simulink model "x64_15l_gonly"  (R2012b)
settings: Solver=VariableStepDiscrete  SolverMode=SingleTasking  StartTime=0.0  StopTime=10.0  RelTol=1e-3
undefined symbols (not defined in the file): gcbh, pfb_coeff_gen_calc, ROACH, xlBlockLoadCallback
libraries: xbsIndex_r4 x10760, casper_library_misc x122, casper_library_delays x52, ox_lib x14, xrbsComm_r4 x8, xps_library x8
(part 1 of 128)
settings Model: Creator=root  LastModifiedBy=jack
settings DataIOCC: SignalLoggingSaveFormat=ModelDataLogs
settings OptimizationCC: InlineParams=on
settings DebuggingCC: FcnCallInpInsideContextMsg=UseLocalSettings  StrictBusMsg=Warning
settings GRTTargetCC: CombineOutputUpdateFcns=off  GRTInterface=on

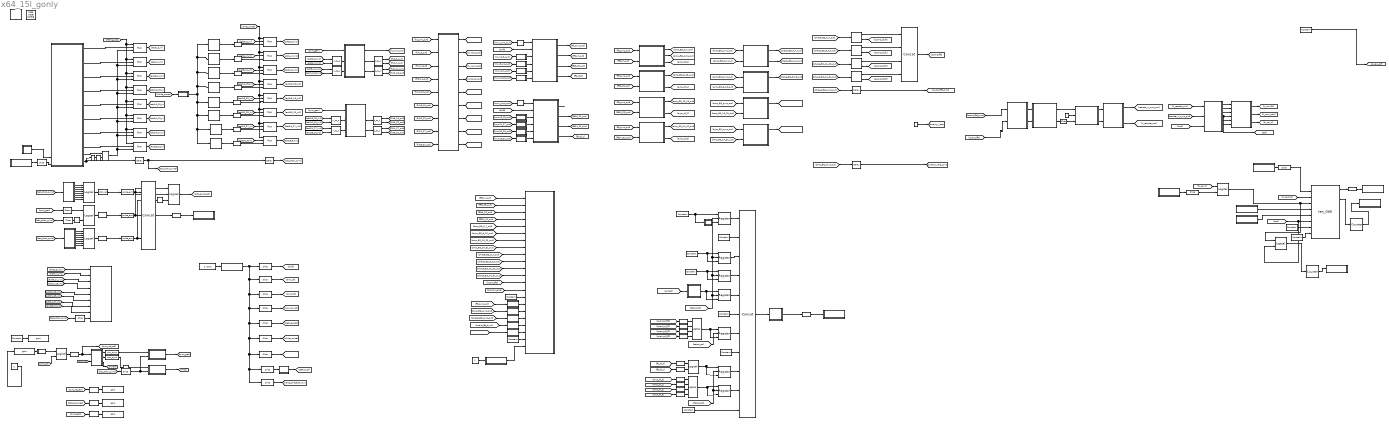
== system x64_15l_gonly ==
  note: revision history:
      |
      | r021a: updated ADC, PFB, FFT blocks
      | removed BF XAUI and logic
      | r021b: get rid of stupid FFTT subsystem
  note: The adc_sync_test reg allows the
      | user to confirm that all 8 ADC chips
      | are syncing together, and that these
      | ADC syncs are arriving the clock before
      | the master sync.
      | If all is going well, the register should
      | show one
  note: bits 0-10: shift
  note: bit 13: xaui tx enable trig
  note: bit 11: sync arm
  note: bit 12: sync rst
  note: We tag on some logic after the
      | sync gen to ensure that a sync pulse
      | arrives the clock before the adc_channel
      | sync, which signifies the arrival
      | of the first multiplexed channel on the
      | adc lines
  note: bit 14: mux in adc chans 4-7 for debug
  note: Data is reordered so that an entire window
      | can be shifted through the FFT
  note: After the FFT, each signal now carries spectra from 8
      | consecutive ADC channels
  note: NFFT = 11
      |
      | NFFT/2 channels
      | 32 (=2^5) ants
      |
      | => 2^(NFFT+4) coeffs
      |
      | 4=2^2 simultaneous streams
      | => 2^(NFFT+2) coeffs per stream
  note: We equalise amplitude and
      | pass data to be quantized to
      | 4 bits and sent to the X engine
      | over XAUI
      | 18 bit precision is maintained so that
      | phase corrections can be added to the
      | data stream going to the fft imaging system.
  note: Phase corrections to the non-FX correlator
      | data streams are implemented here, before quantization
      | to 4 bits takes place
  note: This is the order that will be used by the beamformer+fftt
      | A single freq. channel is repeated  2^(QDR_output_blocksize - 3) times
  note: Whilst the X engine expects groups of a single channel and a single
      | antenna, the fourier imager expects blocks of all antennas * one frequency channel.
  note: [ [0:8:1023] [1:8:1023] [2:8:1023] [3:8:1023]
      | [4:8:1023] [5:8:1023] [6:8:1023] [7:8:1023] ]
  note: Data is tagged with a mcnt number and sync and eof headers.
      | These are later decoded and used for error checking / data ordering
      | in the spatial imager and X-engines
  note: r022a: added MCNT sw reg, compile for library with xBlock SW reg
      | r022b: added white noise generators
      |
      | r023a: 14/03/2011 Changed ADC sync test flags to pulse extend rather than periodically
      | reset registers. Replaced of_reg and snap blocks with status reg from GMRT F-engine
      | and multipurpose snap block from GMRT F-engine. Changed adc power block for power/snap combination.
      | Changed sync period to take into account non 2^N reorder orders in various blocks.
      | 15/03/2011 Black boxed FIR/FFT. Various syntax fixes
  note: bit 15: white noise generator
  note: bit 15: white noise generator rst
  note: ADC overflow
      | Beam Buffer write clash
      | Beam Buffer bad
      | beam buffer valid
      | sync armed
      | beam coeff of
      | fft overflow
      | amp eq overflow
  note: Non 2^N periods:
      | fft mux -- 13
      | QDR transpose -- 11
      | post QDR reorder -- 10
      | reorder 1_ant_a_time -- 7
      | LCM(13,11,10,7) = 10010
  note: bit 19: reset status flags
  note: The FFT interleaves antenna spectra (though blocks of N_FFT/2 channels
      | remain contiguous.
      | The signal description "0_7" here, means the first 7 antennas, in the order:
      | 0,4,1,5,2,6,3,7
      | Similarly, signals named "x_x+7" have the order
      | x,x+4,x+1,x+5,x+2,x+6,x+3,x+7
      | This order needs to be reflected in the arrangement of coefficients
      | in the downstream EQ RAM blocks.
  note: bit 20: Xengine phased input mux
  note: scale inputs down by 2 bits
  " System Generator" : xbsIndex_r4/ System Generator  Tag=genX  xilinxfamily=virtex5  part=xc5vsx95t  speed=-1  package=ff1136  synthesis_tool=XST  clock_wrapper=Clock Enables  directory=./x64_32f_024i_15lg/sysgen  proj_type=Project Navigator  Synth_file=XST Defaults  Impl_file=ISE Defaults  testbench=off  simulink_period=1  sysclk_period=6.25  dcm_input_clock_period=100  incr_netlist=off  trim_vbits=Everywhere in SubSystem  dbl_ovrd=According to Block Masks  core_generation=According to Block Masks  run_coregen=off  deprecated_control=off  eval_field=0  block_type=sysgen
      settings: block_version=11.4
  Concat1 : xbsIndex_r4/Concat  num_inputs=11  dbl_ovrd=off  block_type=concat
  Concat4 : xbsIndex_r4/Concat  num_inputs=4  dbl_ovrd=off  block_type=concat
  Concat6 : xbsIndex_r4/Concat  num_inputs=3  dbl_ovrd=off  block_type=concat
  Constant : xbsIndex_r4/Constant  const=1  gui_display_data_type=Fixed-point  arith_type=Boolean  n_bits=16  bin_pt=14  preci_type=Single  exp_width=8  frac_width=24  explicit_period=on  period=1  equ=P=C  opselect=C  inp2=PCIN>>17  opr=+  inp1=P  carry=CIN  dbl_ovrd=off  block_type=constant
      settings: block_version=11.4
  Constant1 : xbsIndex_r4/Constant  const=0  gui_display_data_type=Fixed-point  arith_type=Signed (2's comp)  n_bits=32  bin_pt=0  preci_type=Single  exp_width=8  frac_width=24  explicit_period=on  period=1  equ=P=C  opselect=C  inp2=PCIN>>17  opr=+  inp1=P  carry=CIN  dbl_ovrd=off  block_type=constant
      settings: block_version=11.4
  Constant13 : Constant
  Constant2 : xbsIndex_r4/Constant  const=1  gui_display_data_type=Fixed-point  arith_type=Boolean  n_bits=16  bin_pt=14  preci_type=Single  exp_width=8  frac_width=24  explicit_period=on  period=1  equ=P=C  opselect=C  inp2=PCIN>>17  opr=+  inp1=P  carry=CIN  dbl_ovrd=off  block_type=constant
      settings: block_version=11.4
  Constant20 : Constant  Value=2^10-1
  Constant3 : Constant
  Constant4 : xbsIndex_r4/Constant  const=0  gui_display_data_type=Boolean  arith_type=Boolean  n_bits=8  bin_pt=0  preci_type=Single  exp_width=8  frac_width=24  explicit_period=on  period=1  equ=P=C  opselect=C  inp2=PCIN>>17  opr=+  inp1=P  carry=CIN  dbl_ovrd=off  block_type=constant
      settings: block_version=11.4
  Constant5 : xbsIndex_r4/Constant  const=1  gui_display_data_type=Boolean  arith_type=Boolean  n_bits=8  bin_pt=0  preci_type=Single  exp_width=8  frac_width=24  explicit_period=on  period=1  equ=P=C  opselect=C  inp2=PCIN>>17  opr=+  inp1=P  carry=CIN  dbl_ovrd=off  block_type=constant
      settings: block_version=11.4
  Constant7 : xbsIndex_r4/Constant  const=0  gui_display_data_type=Fixed-point  arith_type=Boolean  n_bits=8  bin_pt=0  preci_type=Single  exp_width=8  frac_width=24  explicit_period=on  period=1  equ=P=C  opselect=C  inp2=PCIN>>17  opr=+  inp1=P  carry=CIN  dbl_ovrd=off  block_type=constant
      settings: block_version=11.4
  Convert : xbsIndex_r4/Convert  gui_display_data_type=Fixed-point  arith_type=Boolean  n_bits=16  bin_pt=14  float_type=Single  exp_bits=8  fraction_bits=24  quantization=Truncate  overflow=Wrap  en=off  latency=0  dbl_ovrd=off  pipeline=off  block_type=convert
      settings: block_version=11.4
  Convert1 : xbsIndex_r4/Convert  gui_display_data_type=Fixed-point  arith_type=Boolean  n_bits=16  bin_pt=14  float_type=Single  exp_bits=8  fraction_bits=24  quantization=Truncate  overflow=Wrap  en=off  latency=0  dbl_ovrd=off  pipeline=off  block_type=convert
      settings: block_version=11.4
  Convert10 : xbsIndex_r4/Convert  gui_display_data_type=Fixed-point  arith_type=Boolean  n_bits=16  bin_pt=14  float_type=Single  exp_bits=8  fraction_bits=24  quantization=Truncate  overflow=Wrap  en=off  latency=0  dbl_ovrd=off  pipeline=off  block_type=convert
      settings: block_version=11.4
  Convert11 : xbsIndex_r4/Convert  gui_display_data_type=Fixed-point  arith_type=Boolean  n_bits=3  bin_pt=0  float_type=Single  exp_bits=8  fraction_bits=24  quantization=Truncate  overflow=Wrap  en=off  latency=0  dbl_ovrd=off  pipeline=off  block_type=convert
      settings: block_version=11.4
  Convert{2..9,12..13} (10 alike) : xbsIndex_r4/Convert  gui_display_data_type=Boolean  arith_type=Boolean  n_bits=3  bin_pt=0  float_type=Single  exp_bits=8  fraction_bits=24  quantization=Truncate  overflow=Wrap  en=off  latency=0  dbl_ovrd=off  pipeline=off  block_type=convert
      settings: block_version=11.4
  Convert14 : xbsIndex_r4/Convert  gui_display_data_type=Fixed-point  arith_type=Unsigned  n_bits=32  bin_pt=0  float_type=Single  exp_bits=8  fraction_bits=24  quantization=Truncate  overflow=Wrap  en=off  latency=0  dbl_ovrd=off  pipeline=off  block_type=convert
      settings: block_version=11.4
  Convert15 : xbsIndex_r4/Convert  gui_display_data_type=Fixed-point  arith_type=Unsigned  n_bits=32  bin_pt=0  float_type=Single  exp_bits=8  fraction_bits=24  quantization=Truncate  overflow=Wrap  en=off  latency=0  dbl_ovrd=off  pipeline=off  block_type=convert
      settings: block_version=11.4
  Convert16 : xbsIndex_r4/Convert  gui_display_data_type=Fixed-point  arith_type=Unsigned  n_bits=32  bin_pt=0  float_type=Single  exp_bits=8  fraction_bits=24  quantization=Truncate  overflow=Wrap  en=off  latency=0  dbl_ovrd=off  pipeline=off  block_type=convert
      settings: block_version=11.4
  Counter : xbsIndex_r4/Counter  cnt_type=Free Running  cnt_to=Inf  operation=Up  start_count=0  cnt_by_val=1  arith_type=Unsigned  n_bits=32  bin_pt=0  load_pin=off  rst=off  en=on  explicit_period=on  period=1  dbl_ovrd=off  use_behavioral_HDL=off  implementation=Fabric  block_type=counter
  Counter1 : xbsIndex_r4/Counter  cnt_type=Free Running  cnt_to=Inf  operation=Up  start_count=0  cnt_by_val=1  arith_type=Unsigned  n_bits=32  bin_pt=0  load_pin=off  rst=off  en=on  explicit_period=on  period=1  dbl_ovrd=off  use_behavioral_HDL=off  implementation=Fabric  block_type=counter
  Delay{,3..4,8} (4 alike) : xbsIndex_r4/Delay  rst=off  infoeditControl=Selection of Reset will increase slice count due to use of real FFs and instead of SRLs  en=off  latency=1  dbl_ovrd=off  reg_retiming=off  block_type=delay
      settings: block_version=11.4
  Delay1 : xbsIndex_r4/Delay  rst=off  infoeditControl=Selection of Reset will increase slice count due to use of real FFs and instead of SRLs  en=off  latency=3  dbl_ovrd=off  reg_retiming=off  block_type=delay
      settings: block_version=11.4
  Delay2 : xbsIndex_r4/Delay  rst=off  infoeditControl=Selection of Reset will increase slice count due to use of real FFs and instead of SRLs  en=off  latency=3  dbl_ovrd=off  reg_retiming=off  block_type=delay
      settings: block_version=11.4
  Delay5 : xbsIndex_r4/Delay  rst=off  infoeditControl=Selection of Reset will increase slice count due to use of real FFs and instead of SRLs  en=off  latency=2  dbl_ovrd=off  reg_retiming=off  block_type=delay
      settings: block_version=11.4
  Delay6 : xbsIndex_r4/Delay  rst=off  infoeditControl=Selection of Reset will increase slice count due to use of real FFs and instead of SRLs  en=off  latency=3  dbl_ovrd=off  reg_retiming=off  block_type=delay
      settings: block_version=11.4
  Delay7 : xbsIndex_r4/Delay  rst=off  infoeditControl=Selection of Reset will increase slice count due to use of real FFs and instead of SRLs  en=off  latency=2  dbl_ovrd=off  reg_retiming=off  block_type=delay
      settings: block_version=11.4
  Inverter : S-Function  AncestorBlock=xbsIndex_r4/Inverter  LoadFcn=xlBlockLoadCallback(gcbh);  FunctionName=sysgen  Parameters=ptable_  EnableBusSupport=off  mask(Xilinx Inverter Block){infoedit=Bitwise logical negation (one's complement) operator., en_sgadvanced=, en=off, latency=0, dbl_ovrd_sgadvanced=, dbl_ovrd=off, xl_use_area_sgadvanced=, xl_use_area=off, xl_area=[0,0,0,0,0,0,0], has_advanced_control=0, sggui_pos=-1,-1,-1,-1, block_type=inv, block_version=11.4, sg_icon_stat=25,24,1,1,white,blue,0,267846e5,right,, sg_mask_display=|, sg_list_contents=, sg_blockgui_xml=}
      mask sg_mask_display=|
      | fprintf('','COMMENT: begin icon graphics');
      | patch([0 1 1 0 ],[0 0 1 1 ],[0.77 0.82 0.91]);
      | patch([0.24 0.08 0.32 0.08 0.24 0.48 0.56 0.64 0.92 0.72 0.52 0.36 0.6 0.36 0.52 0.72 0.92 0.64 0.56 0.48 0.24 ],[0.125 0.291667 0.541667 0.791667 0.958333 0.958333 0.875 0.958333 0.958333 0.75 0.958333 0.791667 0.541667 0.291667 0.125 0.333333 0.125 0.125 0.208333 0.125 0.125 ],[0.98 0.96 0.92]);
      | plot([0 1 1 0 0 ],[0 0 1 1 0 ]);
      | fprintf('','COMMENT: end icon graphics');
      | fprintf('','COMMENT: begin icon text');
      | color('black');disp('not');
      | fprintf('','COMMENT: end icon text');
      mask prompts: infoedit ""; en_sgadvanced ""; en "Provide enable port"; dbl_ovrd_sgadvanced ""; dbl_ovrd "Override with doubles"; xl_use_area_sgadvanced ""; xl_use_area "Define FPGA area for resource estimation"; xl_area "FPGA area [slices, FFs, BRAMs, LUTs, IOBs, emb. mults, TBUFs]"; has_advanced_control ""; sggui_pos ""; block_type ""; block_version ""; sg_icon_stat ""; sg_mask_display ""; sg_list_contents ""; sg_blockgui_xml ""
      mask help: Bitwise logical negation (one's complement) operator.
      mask init:
      | try
      |   tmp_gcb = gcb;
      |   tmp_gcbh = gcbh;
      |   if (strcmp('SysGenIndex',get_param(bdroot(tmp_gcbh),'tag')) && ~isempty(regexp(bdroot(tmp_gcb), '^xbs', 'once')))
      |     return;
      |   end;
      |   xlMungeMaskParams;
      |   block_config = 'sysgen_blockset:Inverter_config';
      | 
      |   block_type='inv';
      | 
      |   serialized_declarations = '{''dbl_ovrd''=>''Int'',''en''=>''Int'',''latency''=>''Int'',''block_type''=>''String''}';
      |   ptable_ = xlblockprep(get_param(tmp_gcb, 'MaskWSVariables'));
      | catch
      |   global dbgsysgen;
      |   if(~isempty(dbgsysgen) && dbgsysgen)
      |     e = regexprep(lasterr, '\n', '\nError: ');
      |     disp(['Error: While running MaskInit code on block ' tmp_gcb ': ' e]);
      |     error(e);
      |   end
      | end
      settings: CopyFcn=xlBlockMoveCallback(gcbh);  DeleteFcn=xlDestroyGui(gcbh);  ModelCloseFcn=xlDestroyGui(gcbh);  PreSaveFcn=xlBlockPreSaveCallback(gcbh);  PostSaveFcn=xlBlockPostSaveCallback(gcbh);  DestroyFcn=xlDestroyGui(gcbh);  OpenFcn=xlOpenGui(gcbh, 'inv_gui.xml', @xlmagicenablement, -1)  CloseFcn=xlDestroyGui(gcbh);  MoveFcn=xlBlockMoveCallback(gcbh);
      mask Help: eval('');xlDoc('-book','sysgen','-topic','Inverter');
      mask Display:
      | fprintf('','COMMENT: begin icon graphics');
      | patch([0 1 1 0 ],[0 0 1 1 ],[0.77 0.82 0.91]);
      | patch([0.24 0.08 0.32 0.08 0.24 0.48 0.56 0.64 0.92 0.72 0.52 0.36 0.6 0.36 0.52 0.72 0.92 0.64 0.56 0.48 0.24 ],[0.125 0.291667 0.541667 0.791667 0.958333 0.958333 0.875 0.958333 0.958333 0.75 0.958333 0.791667 0.541667 0.291667 0.125 0.333333 0.125 0.125 0.208333 0.125 0.125 ],[0.98 0.96 0.92]);
      | plot([0 1 1 0 0 ],[0 0 1 1 0 ]);
      | fprintf('','COMMENT: end icon graphics');
      | fprintf('','COMMENT: begin icon text');
      | color('black');disp('not');
      | fprintf('','COMMENT: end icon text');
  Inverter1 : S-Function  AncestorBlock=xbsIndex_r4/Inverter  LoadFcn=xlBlockLoadCallback(gcbh);  FunctionName=sysgen  Parameters=ptable_  EnableBusSupport=off  mask(Xilinx Inverter Block){infoedit=Bitwise logical negation (one's complement) operator., en_sgadvanced=, en=off, latency=0, dbl_ovrd_sgadvanced=, dbl_ovrd=off, xl_use_area_sgadvanced=, xl_use_area=off, xl_area=[0,0,0,0,0,0,0], has_advanced_control=0, sggui_pos=-1,-1,-1,-1, block_type=inv, block_version=11.4, sg_icon_stat=25,24,1,1,white,blue,0,267846e5,right,, sg_mask_display=|, sg_list_contents=, sg_blockgui_xml=}
      mask sg_mask_display=|
      | fprintf('','COMMENT: begin icon graphics');
      | patch([0 1 1 0 ],[0 0 1 1 ],[0.77 0.82 0.91]);
      | patch([0.24 0.08 0.32 0.08 0.24 0.48 0.56 0.64 0.92 0.72 0.52 0.36 0.6 0.36 0.52 0.72 0.92 0.64 0.56 0.48 0.24 ],[0.125 0.291667 0.541667 0.791667 0.958333 0.958333 0.875 0.958333 0.958333 0.75 0.958333 0.791667 0.541667 0.291667 0.125 0.333333 0.125 0.125 0.208333 0.125 0.125 ],[0.98 0.96 0.92]);
      | plot([0 1 1 0 0 ],[0 0 1 1 0 ]);
      | fprintf('','COMMENT: end icon graphics');
      | fprintf('','COMMENT: begin icon text');
      | color('black');disp('not');
      | fprintf('','COMMENT: end icon text');
      mask prompts: infoedit ""; en_sgadvanced ""; en "Provide enable port"; dbl_ovrd_sgadvanced ""; dbl_ovrd "Override with doubles"; xl_use_area_sgadvanced ""; xl_use_area "Define FPGA area for resource estimation"; xl_area "FPGA area [slices, FFs, BRAMs, LUTs, IOBs, emb. mults, TBUFs]"; has_advanced_control ""; sggui_pos ""; block_type ""; block_version ""; sg_icon_stat ""; sg_mask_display ""; sg_list_contents ""; sg_blockgui_xml ""
      mask help: Bitwise logical negation (one's complement) operator.
      mask init: same as x64_15l_gonly/Inverter
      settings: CopyFcn=xlBlockMoveCallback(gcbh);  DeleteFcn=xlDestroyGui(gcbh);  ModelCloseFcn=xlDestroyGui(gcbh);  PreSaveFcn=xlBlockPreSaveCallback(gcbh);  PostSaveFcn=xlBlockPostSaveCallback(gcbh);  DestroyFcn=xlDestroyGui(gcbh);  OpenFcn=xlOpenGui(gcbh, 'inv_gui.xml', @xlmagicenablement, -1)  CloseFcn=xlDestroyGui(gcbh);  MoveFcn=xlBlockMoveCallback(gcbh);
      mask Help: eval('');xlDoc('-book','sysgen','-topic','Inverter');
      mask Display:
      | fprintf('','COMMENT: begin icon graphics');
      | patch([0 1 1 0 ],[0 0 1 1 ],[0.77 0.82 0.91]);
      | patch([0.24 0.08 0.32 0.08 0.24 0.48 0.56 0.64 0.92 0.72 0.52 0.36 0.6 0.36 0.52 0.72 0.92 0.64 0.56 0.48 0.24 ],[0.125 0.291667 0.541667 0.791667 0.958333 0.958333 0.875 0.958333 0.958333 0.75 0.958333 0.791667 0.541667 0.291667 0.125 0.333333 0.125 0.125 0.208333 0.125 0.125 ],[0.98 0.96 0.92]);
      | plot([0 1 1 0 0 ],[0 0 1 1 0 ]);
      | fprintf('','COMMENT: end icon graphics');
      | fprintf('','COMMENT: begin icon text');
      | color('black');disp('not');
      | fprintf('','COMMENT: end icon text');
  Logical : xbsIndex_r4/Logical  logical_function=AND  inputs=2  en=off  latency=0  precision=Full  arith_type=Unsigned  n_bits=16  bin_pt=0  align_bp=on  dbl_ovrd=off  block_type=logical
  Logical1 : xbsIndex_r4/Logical  logical_function=XOR  inputs=8  en=off  latency=1  precision=Full  arith_type=Unsigned  n_bits=8  bin_pt=2  align_bp=on  dbl_ovrd=off  block_type=logical
      settings: xl_area=[0, 0, 0, 0, 0, 0, 0]
  Logical2 : xbsIndex_r4/Logical  logical_function=AND  inputs=2  en=off  latency=1  precision=Full  arith_type=Unsigned  n_bits=8  bin_pt=2  align_bp=on  dbl_ovrd=off  block_type=logical
      settings: xl_area=[0, 0, 0, 0, 0, 0, 0]
  Logical3 : xbsIndex_r4/Logical  logical_function=OR  inputs=2  en=off  latency=1  precision=Full  arith_type=Unsigned  n_bits=16  bin_pt=0  align_bp=on  dbl_ovrd=off  block_type=logical
      settings: block_version=11.4
  Logical4 : xbsIndex_r4/Logical  logical_function=OR  inputs=4  en=off  latency=1  precision=Full  arith_type=Unsigned  n_bits=16  bin_pt=0  align_bp=on  dbl_ovrd=off  block_type=logical
      settings: block_version=11.4
  Logical5 : xbsIndex_r4/Logical  logical_function=OR  inputs=4  en=off  latency=1  precision=Full  arith_type=Unsigned  n_bits=16  bin_pt=0  align_bp=on  dbl_ovrd=off  block_type=logical
      settings: block_version=11.4
  Logical6 : xbsIndex_r4/Logical  logical_function=AND  inputs=8  en=off  latency=1  precision=Full  arith_type=Unsigned  n_bits=8  bin_pt=2  align_bp=on  dbl_ovrd=off  block_type=logical
      settings: xl_area=[0, 0, 0, 0, 0, 0, 0]
  Logical7 : xbsIndex_r4/Logical  logical_function=OR  inputs=2  en=off  latency=1  precision=Full  arith_type=Unsigned  n_bits=8  bin_pt=2  align_bp=on  dbl_ovrd=off  block_type=logical
      settings: xl_area=[0, 0, 0, 0, 0, 0, 0]
  Logical8 : xbsIndex_r4/Logical  logical_function=OR  inputs=3  en=off  latency=1  precision=Full  arith_type=Unsigned  n_bits=8  bin_pt=2  align_bp=on  dbl_ovrd=off  block_type=logical
      settings: xl_area=[0, 0, 0, 0, 0, 0, 0]
  Logical9 : xbsIndex_r4/Logical  logical_function=AND  inputs=2  en=off  latency=0  precision=Full  arith_type=Unsigned  n_bits=16  bin_pt=0  align_bp=on  dbl_ovrd=off  block_type=logical
  Mux{1..16} (16 alike) : xbsIndex_r4/Mux  inputs=2  en=off  latency=1  precision=Full  arith_type=Unsigned  n_bits=16  bin_pt=14  quantization=Truncate  overflow=Wrap  dbl_ovrd=off  block_type=mux
      settings: block_version=11.4
  Register : xbsIndex_r4/Register  init=0  rst=off  en=on  dbl_ovrd=off  block_type=register
      settings: block_version=11.4
  Regster{1..6,8} (7 alike) : xbsIndex_r4/Register  init=0  rst=on  en=on  dbl_ovrd=off  block_type=register
      settings: block_version=11.4
  Reinterpret{1..8} (8 alike) : xbsIndex_r4/Reinterpret  force_arith_type=off  arith_type=Unsigned  force_bin_pt=on  bin_pt=11  block_type=reinterpret
      settings: infoedit="Changes signal type without altering the binary representation.   You can changed the signal between signed and unsigned, and relocate the binary point.<br><br>Hardware notes: In hardware this block costs nothing.<br><br>Example:  Suppose the input is 6 bits wide, signed, with 2 fractional bits, and the output is forced to unsigned with 0 fractional bits.  Then an input of -2.0 (1110.00 in binary 2's complement) becomes an output of 56 (111000 in binary)."
  Slice : xbsIndex_r4/Slice  nbits=11  boolean_output=off  mode=Lower Bit Location + Width  bit1=0  base1=MSB of Input  bit0=0  base0=LSB of Input  dbl_ovrd=off  block_type=slice
  Slice{1,3,7,9} (4 alike) : xbsIndex_r4/Slice  nbits=1  boolean_output=on  mode=Lower Bit Location + Width  bit1=0  base1=MSB of Input  bit0=0  base0=LSB of Input  dbl_ovrd=off  block_type=slice
  Slice10 : xbsIndex_r4/Slice  nbits=1  boolean_output=on  mode=Lower Bit Location + Width  bit1=0  base1=MSB of Input  bit0=0  base0=MSB of Input  dbl_ovrd=off  block_type=slice
  Slice11 : xbsIndex_r4/Slice  nbits=1  boolean_output=on  mode=Lower Bit Location + Width  bit1=0  base1=MSB of Input  bit0=14  base0=LSB of Input  dbl_ovrd=off  block_type=slice
  Slice12 : xbsIndex_r4/Slice  nbits=1  boolean_output=on  mode=Lower Bit Location + Width  bit1=0  base1=MSB of Input  bit0=13  base0=LSB of Input  dbl_ovrd=off  block_type=slice
  Slice13 : xbsIndex_r4/Slice  nbits=32  boolean_output=off  mode=Lower Bit Location + Width  bit1=0  base1=MSB of Input  bit0=0  base0=LSB of Input  dbl_ovrd=off  block_type=slice
  Slice14 : xbsIndex_r4/Slice  nbits=1  boolean_output=on  mode=Lower Bit Location + Width  bit1=0  base1=MSB of Input  bit0=15  base0=LSB of Input  dbl_ovrd=off  block_type=slice
  Slice15 : xbsIndex_r4/Slice  nbits=1  boolean_output=on  mode=Lower Bit Location + Width  bit1=0  base1=MSB of Input  bit0=15  base0=LSB of Input  dbl_ovrd=off  block_type=slice
  Slice16 : xbsIndex_r4/Slice  nbits=1  boolean_output=on  mode=Lower Bit Location + Width  bit1=0  base1=MSB of Input  bit0=20  base0=LSB of Input  dbl_ovrd=off  block_type=slice
  Slice2 : xbsIndex_r4/Slice  nbits=1  boolean_output=on  mode=Lower Bit Location + Width  bit1=0  base1=MSB of Input  bit0=12  base0=LSB of Input  dbl_ovrd=off  block_type=slice
  Slice22 : xbsIndex_r4/Slice  nbits=1  boolean_output=on  mode=Lower Bit Location + Width  bit1=0  base1=MSB of Input  bit0=19  base0=LSB of Input  dbl_ovrd=off  block_type=slice
  Slice4 : xbsIndex_r4/Slice  nbits=1  boolean_output=on  mode=Lower Bit Location + Width  bit1=0  base1=MSB of Input  bit0=11  base0=LSB of Input  dbl_ovrd=off  block_type=slice
  Slice5 : xbsIndex_r4/Slice  nbits=3  boolean_output=on  mode=Lower Bit Location + Width  bit1=0  base1=MSB of Input  bit0=0  base0=LSB of Input  dbl_ovrd=off  block_type=slice
  Slice8 : xbsIndex_r4/Slice  nbits=3  boolean_output=on  mode=Lower Bit Location + Width  bit1=0  base1=MSB of Input  bit0=0  base0=LSB of Input  dbl_ovrd=off  block_type=slice
  White Gaussian Noise Generator : xrbsComm_r4/White Gaussian  Noise Generator  seed=33960
  White Gaussian Noise Generator1 : xrbsComm_r4/White Gaussian  Noise Generator  seed=25231
  White Gaussian Noise Generator2 : xrbsComm_r4/White Gaussian  Noise Generator  seed=1867
  White Gaussian Noise Generator3 : xrbsComm_r4/White Gaussian  Noise Generator  seed=39006
  White Gaussian Noise Generator4 : xrbsComm_r4/White Gaussian  Noise Generator  seed=13142
  White Gaussian Noise Generator5 : xrbsComm_r4/White Gaussian  Noise Generator  seed=42291
  White Gaussian Noise Generator6 : xrbsComm_r4/White Gaussian  Noise Generator  seed=7242
  White Gaussian Noise Generator7 : xrbsComm_r4/White Gaussian  Noise Generator  seed=31337
  XSG_core_config : xps_library/XSG core config  Tag=xps:xsg  hw_sys=ROACH:sx95t  clk_src=adc0_clk  ROACH_clk_src=adc0_clk  ROACH2_clk_src=adc0_clk  clk_rate=160  sample_period=1  synthesis_tool=XST
  a : Subsystem  mask{n_fft=11, n_adc=32, n_streams=3}
      mask prompts: n_fft "FFT size (2^?)"; n_adc "Number of adc channels?"; n_streams "Number of adc streams (2^?)"
      mask init:
      | %part_reorder = [0:n_adc:(2^(n_fft-n_streams))*n_adc-3]
      | %reorder = [];
      | %for adc_chan = [0:n_adc-1]
      | %    reorder = [reorder,[part_reorder]+adc_chan];
      | %end
      | 
      | part_reorder = [0:4:2^(n_fft+2)-1];
      | lp = size(part_reorder,2);
      | reorder = zeros(1,lp*4);
      | for m = [0:3]
      |     reorder(m*lp+1:(m+1)*lp) = part_reorder+m;
      | end
      | 
      | s = tostring(reorder,4)
      | set_param([gcb, '/r'], 'map', s);
  adc_sim_sync : Subsystem
  adc_spi_ctrl : Subsystem  Tag=xps:sw_reg  AncestorBlock=xps_library/software register  mask(swreg){mode=one value, io_dir=From Processor, io_delay=0, sample_period=1, names=reg, bitwidths=32, arith_types=0, bin_pts=0, show_format=off}
      mask prompts: io_dir "I/O direction"; io_delay "I/O delay"; sample_period "Sample period"; names "Name:"; bitwidths "Bitwidth:"; arith_types "Type (ufix=0, fix=1, bool=2):"; bin_pts "Binary pt:"; show_format "Print format string?"
      mask init:
      | swreg_init(gcb)
      settings: AttributesFormatString=1input
      mask TypeOptions mode: one value | fields of equal size | fields of arbitrary size
      mask Callback mode: swreg_cb(gcb);
      mask TypeOptions io_dir: To Processor | From Processor
      mask Callback io_dir:
      | mask_enables = get_param(gcb, 'MaskEnables');
      | mask_names = get_param(gcb, 'MaskNames');
      | if strcmp(get_param(gcb, 'io_dir'), 'To Processor'),
      |     mask_enables{ismember(mask_names, 'sample_period')} = 'off';
      | else
      |     mask_enables{ismember(mask_names, 'sample_period')} = 'on';
      | end
      | set_param(gcb, 'MaskEnables', mask_enables);
      mask Callback bitwidths:
      | blk = gcb;
      | mode = get_param(blk, 'mode');
      | current_widths = eval(get_param(blk, 'bitwidths'));
      | if (strcmp(mode, 'one value') || strcmp(mode, 'fields of equal size')) && (length(current_widths) > 1),
      |     error('Only one width may be specified for this mode.');
      | elseif strcmp(mode, 'fields of arbitrary size')
      |     current_names = textscan(strtrim(strrep(strrep(get_param(blk, 'names'), ']', ''), '[', '')), '%s');
      |     current_names = current_names{1};
      |     numios = length(current_names);
      |     if length(current_widths) ~= numios,
      |         error('%d field names specified, but %d widths?', numios, length(current_widths));
      |     end
      | end
      | total_width = 0;
      | for ctr = 1 : length(current_widths),
      |     total_width = total_width + current_widths(ctr);
      | end
      | if total_width > 32,
      |     error('Total width must be 32 or less, set to %d.', total_width);
      | end
      mask Callback arith_types:
      | blk = gcb;
      | mode = get_param(blk, 'mode');
      | current_types = eval(get_param(blk, 'arith_types'));
      | numios = length(current_types);
      | if (strcmp(mode, 'one value') || strcmp(mode, 'fields of equal size')) && (length(current_types) > 1),
      |     error('Only one type may be specified for this mode.');
      | elseif strcmp(mode, 'fields of arbitrary size')
      |     current_names = textscan(strtrim(strrep(strrep(get_param(blk, 'names'), ']', ''), '[', '')), '%s');
      |     current_names = current_names{1};
      |     numios = length(current_names);
      |     if length(current_types) ~= numios,
      |         error('%d field names specified, but %d types?', numios, length(current_types));
      |     end
      | end
      | problem = 0;
      | for ctr = 1 : numios,
      |     t = current_types(ctr);
      |     if (t < 0) || (t > 2),
      |         problem = t;
      |         ctr = numios + 1;
      |     end
      | end
      | if problem ~= 0,
      |     error('Type cannot be %i, must be 0, 1 or 2.', problem);
      | end
      mask Callback bin_pts:
      | blk = gcb;
      | mode = get_param(blk, 'mode');
      | current_bins = eval(get_param(blk, 'bin_pts'));
      | if (strcmp(mode, 'one value') || strcmp(mode, 'fields of equal size')) && (length(current_bins) > 1),
      |     error('Only one binary pt may be specified for this mode.');
      | elseif strcmp(mode, 'fields of arbitrary size')
      |     current_names = textscan(strtrim(strrep(strrep(get_param(blk, 'names'), ']', ''), '[', '')), '%s');
      |     current_names = current_names{1};
      |     numios = length(current_names);
      |     if length(current_bins) ~= numios,
      |         error('%d field names specified, but %d binary pts?', numios, length(current_bins));
      |     end
      | end
  adc_sw : Subsystem
  adc_sync_align : Subsystem
  adc_sync_align1 : Subsystem
  adc_sync_test : Subsystem  Tag=xps:sw_reg  mask{io_dir=To Processor, arith_type=Unsigned, bitwidth=32, bin_pt=0, sample_period=1, latency=0}
      mask prompts: io_dir "I/O direction"; arith_type "Data Type"; bitwidth "Data bitwidth"; bin_pt "Data binary point"; sample_period "Sample period"
      mask init:
      | gw_name = clear_name(gcb);
      | config.source = str2func('software_register_init');
      | config.toplevel = gcb;
      | xBlock( config, {io_dir, arith_type, bitwidth, bin_pt, ... 
      |     sample_period, gw_name, latency});
      mask TypeOptions io_dir: From Processor | To Processor
      mask TypeOptions arith_type: Unsigned | Signed  (2's comp)
  amp_EQ0 : Subsystem  mask{N=11-1+5-2 -1, bram_lat=2, mult_lat=3, add_lat=2}
      mask prompts: N "number of coefficients (2^?)"; bram_lat "bram latency"; mult_lat "multiplier latency"; add_lat "adder latency"
      mask init:
      | set_param([gcb, '/coeff_bram'], 'addr_width', num2str(N));
  amp_EQ1 : Subsystem  mask{N=11-1+5-2 -1, bram_lat=2, mult_lat=3, add_lat=2}
      mask prompts: N "number of coefficients (2^?)"; bram_lat "bram latency"; mult_lat "multiplier latency"; add_lat "adder latency"
      mask init:
      | set_param([gcb, '/coeff_bram'], 'addr_width', num2str(N));
  amp_EQ2 : Subsystem  mask{N=11-1+5-2 -1, bram_lat=2, mult_lat=3, add_lat=2}
      mask prompts: N "number of coefficients (2^?)"; bram_lat "bram latency"; mult_lat "multiplier latency"; add_lat "adder latency"
      mask init:
      | set_param([gcb, '/coeff_bram'], 'addr_width', num2str(N));
  amp_EQ3 : Subsystem  mask{N=11-1+5-2 -1, bram_lat=2, mult_lat=3, add_lat=2}
      mask prompts: N "number of coefficients (2^?)"; bram_lat "bram latency"; mult_lat "multiplier latency"; add_lat "adder latency"
      mask init:
      | set_param([gcb, '/coeff_bram'], 'addr_width', num2str(N));
  bus_expand : Subsystem  AncestorBlock=casper_library_flow_control/bus_expand  mask(bus_expand){mode=divisions of equal size, outputNum=8, outputWidth=1, outputBinaryPt=0, outputArithmeticType=2, show_format=off, outputToWorkspace=off, variablePrefix=out, outputToModelAsWell=on}
      mask prompts: outputNum "Number of outputs:"; outputWidth "Output width:"; outputBinaryPt "Output binary point position:"; outputArithmeticType "Output arithmetic type (ufix=0, fix=1, bool=2):"; show_format "Print format string?"; outputToWorkspace "Output to workspace?"; variablePrefix "Variable name prefix:"; outputToModelAsWell "Output to model as well?"
      mask help:
      | Expands a 'bus' made using a bus_create or Xilinx
      | concat block.
      | The input will be divided into the specified number
      | of outputs with the specified arithmetic types.
      | Divisions are made from most significant bit.
      mask init:
      | bus_expand_init(gcb,...
      |     'mode', mode, ...
      |     'outputNum', outputNum, ...
      |     'outputWidth', outputWidth, ...
      |     'outputBinaryPt', outputBinaryPt, ...
      |     'outputArithmeticType', outputArithmeticType, ...
      |     'show_format', show_format, ...
      |     'outputToWorkspace', outputToWorkspace, ...
      |     'variablePrefix', variablePrefix, ...
      |     'outputToModelAsWell', outputToModelAsWell);
      settings: AttributesFormatString=8 outputs
      mask TypeOptions mode: divisions of equal size | divisions of arbitrary size
      mask Callback mode: bus_expand_callback();
      mask Callback outputWidth: bus_expand_callback();
      mask Callback outputToWorkspace: bus_expand_callback();
  bus_expand1 : Subsystem  AncestorBlock=casper_library_flow_control/bus_expand  mask(bus_expand){mode=divisions of equal size, outputNum=8, outputWidth=1, outputBinaryPt=0, outputArithmeticType=2, show_format=off, outputToWorkspace=off, variablePrefix=out, outputToModelAsWell=on}
      mask prompts: outputNum "Number of outputs:"; outputWidth "Output width:"; outputBinaryPt "Output binary point position:"; outputArithmeticType "Output arithmetic type (ufix=0, fix=1, bool=2):"; show_format "Print format string?"; outputToWorkspace "Output to workspace?"; variablePrefix "Variable name prefix:"; outputToModelAsWell "Output to model as well?"
      mask help:
      | Expands a 'bus' made using a bus_create or Xilinx
      | concat block.
      | The input will be divided into the specified number
      | of outputs with the specified arithmetic types.
      | Divisions are made from most significant bit.
      mask init: same as x64_15l_gonly/bus_expand
      settings: AttributesFormatString=8 outputs
      mask TypeOptions mode: divisions of equal size | divisions of arbitrary size
      mask Callback mode: bus_expand_callback();
      mask Callback outputWidth: bus_expand_callback();
      mask Callback outputToWorkspace: bus_expand_callback();
  c_to_ri{,1..3} (4 alike) : casper_library_misc/c_to_ri  n_bits=18  bin_pt=17
  chan_reorder : Subsystem  mask{partial_init=[0 512], n_chan=1024}
      mask prompts: partial_init "Partial Reorder"; n_chan "Number of channels"
      mask init:
      | pr = partial_init;
      | 
      | r = []
      | for i=[0:(n_chan/2)-1]
      |     r=[r, pr+i];
      | end
      | 
      | r
      | 
      | set_param([gcb, '/reorder'], 'map', tostring(r));
  ctrl_sw : Subsystem  Tag=xps:sw_reg  AncestorBlock=xps_library/software register  mask(swreg){mode=one value, io_dir=From Processor, io_delay=0, sample_period=1, names=reg, bitwidths=32, arith_types=0, bin_pts=0, show_format=off}
      mask prompts: io_dir "I/O direction"; io_delay "I/O delay"; sample_period "Sample period"; names "Name:"; bitwidths "Bitwidth:"; arith_types "Type (ufix=0, fix=1, bool=2):"; bin_pts "Binary pt:"; show_format "Print format string?"
      mask init:
      | swreg_init(gcb)
      settings: AttributesFormatString=1input
      mask TypeOptions mode: one value | fields of equal size | fields of arbitrary size
      mask Callback mode: swreg_cb(gcb);
      mask TypeOptions io_dir: To Processor | From Processor
      mask Callback io_dir:
      | mask_enables = get_param(gcb, 'MaskEnables');
      | mask_names = get_param(gcb, 'MaskNames');
      | if strcmp(get_param(gcb, 'io_dir'), 'To Processor'),
      |     mask_enables{ismember(mask_names, 'sample_period')} = 'off';
      | else
      |     mask_enables{ismember(mask_names, 'sample_period')} = 'on';
      | end
      | set_param(gcb, 'MaskEnables', mask_enables);
      mask Callback bitwidths:
      | blk = gcb;
      | mode = get_param(blk, 'mode');
      | current_widths = eval(get_param(blk, 'bitwidths'));
      | if (strcmp(mode, 'one value') || strcmp(mode, 'fields of equal size')) && (length(current_widths) > 1),
      |     error('Only one width may be specified for this mode.');
      | elseif strcmp(mode, 'fields of arbitrary size')
      |     current_names = textscan(strtrim(strrep(strrep(get_param(blk, 'names'), ']', ''), '[', '')), '%s');
      |     current_names = current_names{1};
      |     numios = length(current_names);
      |     if length(current_widths) ~= numios,
      |         error('%d field names specified, but %d widths?', numios, length(current_widths));
      |     end
      | end
      | total_width = 0;
      | for ctr = 1 : length(current_widths),
      |     total_width = total_width + current_widths(ctr);
      | end
      | if total_width > 32,
      |     error('Total width must be 32 or less, set to %d.', total_width);
      | end
      mask Callback arith_types:
      | blk = gcb;
      | mode = get_param(blk, 'mode');
      | current_types = eval(get_param(blk, 'arith_types'));
      | numios = length(current_types);
      | if (strcmp(mode, 'one value') || strcmp(mode, 'fields of equal size')) && (length(current_types) > 1),
      |     error('Only one type may be specified for this mode.');
      | elseif strcmp(mode, 'fields of arbitrary size')
      |     current_names = textscan(strtrim(strrep(strrep(get_param(blk, 'names'), ']', ''), '[', '')), '%s');
      |     current_names = current_names{1};
      |     numios = length(current_names);
      |     if length(current_types) ~= numios,
      |         error('%d field names specified, but %d types?', numios, length(current_types));
      |     end
      | end
      | problem = 0;
      | for ctr = 1 : numios,
      |     t = current_types(ctr);
      |     if (t < 0) || (t > 2),
      |         problem = t;
      |         ctr = numios + 1;
      |     end
      | end
      | if problem ~= 0,
      |     error('Type cannot be %i, must be 0, 1 or 2.', problem);
      | end
      mask Callback bin_pts:
      | blk = gcb;
      | mode = get_param(blk, 'mode');
      | current_bins = eval(get_param(blk, 'bin_pts'));
      | if (strcmp(mode, 'one value') || strcmp(mode, 'fields of equal size')) && (length(current_bins) > 1),
      |     error('Only one binary pt may be specified for this mode.');
      | elseif strcmp(mode, 'fields of arbitrary size')
      |     current_names = textscan(strtrim(strrep(strrep(get_param(blk, 'names'), ']', ''), '[', '')), '%s');
      |     current_names = current_names{1};
      |     numios = length(current_names);
      |     if length(current_bins) ~= numios,
      |         error('%d field names specified, but %d binary pts?', numios, length(current_bins));
      |     end
      | end
  edge_detect : Subsystem  AncestorBlock=casper_library_misc/edge_detect  mask(edge_detect){edge=Rising, polarity=Active High, x_in=[0 0.08 0.08 0.16 0.16 0.24 0.24 0.32 0.32 0.4], y_in=[-1 -1  1  1  1  1  1  1  1  1], x_out=[0.6 0.68 0.68 0.76 0.76 0.84 0.84 0.92 0.92 1], y_out=[-1 -1  1  1 -1 -1 -1 -1 -1 -1]}
      mask prompts: edge "Edge Type"; polarity "Output Polarity"; x_in "Input X Positions"; y_in "Input Y Positions"; x_out "Output X Positions"; y_out "Output Y Positions"
      mask help: Output is active for one-cycle after each edge of the specified type (i.e. rising, falling or both).
      mask init:
      | edge_detect_init(gcb,...
      |     'edge',edge,...
      |     'polarity',polarity,...
      |     'x_in',x_in,...
      |     'x_out',x_out,...
      |     'y_in',y_in,...
      |     'y_out',y_out);
      | 
      | x_in_num=str2num(getfield(getfield(get_param(gcb,'UserData'),'parameters'),'x_in'));
      | x_out_num=str2num(getfield(getfield(get_param(gcb,'UserData'),'parameters'),'x_out'));
      | y_in_num=str2num(getfield(getfield(get_param(gcb,'UserData'),'parameters'),'y_in'));
      | y_out_num=str2num(getfield(getfield(get_param(gcb,'UserData'),'parameters'),'y_out'));
      settings: AttributesFormatString=|
      | rising edges
      | active high
      mask Help: Output is active for one-cycle after each edge of the specified type (i.e. rising, falling, or both).  Latency is zero.
      mask TypeOptions edge: Rising | Falling | Both
      mask TypeOptions polarity: Active High | Active Low
      mask Display:
      | plot(x_in_num,0.5+y_in_num*0.2);
      | plot(x_out_num,0.5+y_out_num*0.2);
  ext{1,3..5,22} (5 alike) : casper_library_misc/pulse_ext  pulse_len=2^25
  ext2 : casper_library_misc/pulse_ext  pulse_len=4
  fft_biplex_real_2x1 : Subsystem  Tag=casper:fft_biplex_real_2x  AncestorBlock=casper_library_ffts/fft_biplex_real_2x  mask(fft_biplex_real_2x){n_inputs=1, FFTSize=11, input_bit_width=18, bin_pt=17, coeff_bit_width=18, async=off, add_latency=1, add_latency_twiddles=0, mult_latency=3, bram_latency=2, conv_latency=2, conv_latency_twiddles=0, quantization=Round  (unbiased: +/- Inf), overflow=Wrap, delays_bit_limit=8, coeffs_bit_limit=8, coeff_sharing=on, coeff_decimation=on, max_fanout=4, mult_spec=1, bitgrowth=off, max_bits=19, hardcode_shifts=off, shift_schedule=[1                                      1], dsp48_adders=off, conv_imp_twiddles=Fabric, conv_imp=Fabric}
      mask prompts: n_inputs "Number simultaneous inputs (4*?)"; FFTSize "Size of FFT: (2^? pts)"; input_bit_width "Input bit width"; bin_pt "Input binary point"; coeff_bit_width "Coefficient Bit Width"; async "Asynchronous operation"; add_latency "Add Latency"; add_latency_twiddles "Add Latency (in twiddles)"; mult_latency "Mult Latency"; bram_latency "BRAM Latency"; conv_latency "Convert latency"; conv_latency_twiddles "Convert latency (in twiddles)"; quantization "Quantization Behavior"; overflow "Overflow Behavior"; delays_bit_limit "Number bits above which to implement stage's delays in BRAM (2^? bits)"; coeffs_bit_limit "Number bits above which to store stage's coefficients in BRAM (2^? bits)"; coeff_sharing "BRAM sharing in coeff storage"; coeff_decimation "Store a fraction of coeff factors where useful"; max_fanout "Maximum fanout"; mult_spec "Multiplier impl. (0=core, 1=embedded, 2=behavioural) (left=1st stage, or just one value)"; bitgrowth "Bit growth instead of shifting"; max_bits "Max bits to growth to"; hardcode_shifts "Hardcode shift schedule"; shift_schedule "Shift schedule"; dsp48_adders "DSP48 adders in butterfly"; conv_imp_twiddles "Convert implementation in twiddles"; conv_imp "Convert implementation"
      mask help: A real-sampled biplex FFT, with output demuxed by 2.
      mask init:
      | fft_biplex_real_2x_init(gcb, ...
      |     'n_inputs', n_inputs, ...
      |     'FFTSize', FFTSize, ...
      |     'input_bit_width', input_bit_width, ... 
      |     'bin_pt', bin_pt, ...
      |     'coeff_bit_width', coeff_bit_width, ...
      |     'async', async, ...
      |     'add_latency', add_latency, ...
      |     'add_latency_twiddles', add_latency_twiddles, ...
      |     'mult_latency', mult_latency, ...
      |     'bram_latency', bram_latency, ...
      |     'conv_latency', conv_latency, ...
      |     'conv_latency_twiddles', conv_latency_twiddles, ...
      |     'quantization', quantization, ...
      |     'overflow', overflow, ...
      |     'delays_bit_limit', delays_bit_limit, ...
      |     'coeffs_bit_limit', coeffs_bit_limit, ...
      |     'coeff_sharing', coeff_sharing, ...
      |     'coeff_decimation', coeff_decimation, ...
      |     'max_fanout', max_fanout, ...
      |     'mult_spec', mult_spec, ...
      |     'bitgrowth', bitgrowth, ...
      |     'max_bits', max_bits, ...
      |     'hardcode_shifts', hardcode_shifts, ...
      |     'shift_schedule', shift_schedule, ...
      |     'dsp48_adders', dsp48_adders, ...
      |     'conv_imp_twiddles', conv_imp_twiddles, ...
      |     'conv_imp', conv_imp);
      settings: AttributesFormatString=|
      | 11 stages
      | [18,18]
      | Round  (unbiased: +/- Inf)
      | Wrap
      mask Help: eval('xlWeb(''http://casper.berkeley.edu/wiki/Fft_biplex_real_2x'')')
      mask TypeOptions quantization: Truncate | Round  (unbiased: +/- Inf) | Round  (unbiased: Even Values)
      mask TypeOptions overflow: Wrap | Saturate | Error
      mask Callback hardcode_shifts:
      | hardcode_shifts = get_param(gcb, 'hardcode_shifts');
      | set_param_state(gcb, 'shift_schedule', hardcode_shifts);
      mask Callback dsp48_adders: fft_callback_dsp48_adders(gcb);
      mask TypeOptions conv_imp_twiddles: Fabric | DSP48 | Behavioural | Xilinx Cast Block
      mask TypeOptions conv_imp: Fabric | DSP48 | Behavioural | Xilinx Cast Block
  fft_biplex_real_2x2 : Subsystem  Tag=casper:fft_biplex_real_2x  AncestorBlock=casper_library_ffts/fft_biplex_real_2x  mask(fft_biplex_real_2x){n_inputs=1, FFTSize=11, input_bit_width=18, bin_pt=17, coeff_bit_width=18, async=off, add_latency=1, add_latency_twiddles=0, mult_latency=3, bram_latency=2, conv_latency=2, conv_latency_twiddles=0, quantization=Round  (unbiased: +/- Inf), overflow=Wrap, delays_bit_limit=8, coeffs_bit_limit=8, coeff_sharing=on, coeff_decimation=on, max_fanout=4, mult_spec=1, bitgrowth=off, max_bits=19, hardcode_shifts=off, shift_schedule=[1                                      1], dsp48_adders=off, conv_imp_twiddles=Fabric, conv_imp=Fabric}
      mask prompts: n_inputs "Number simultaneous inputs (4*?)"; FFTSize "Size of FFT: (2^? pts)"; input_bit_width "Input bit width"; bin_pt "Input binary point"; coeff_bit_width "Coefficient Bit Width"; async "Asynchronous operation"; add_latency "Add Latency"; add_latency_twiddles "Add Latency (in twiddles)"; mult_latency "Mult Latency"; bram_latency "BRAM Latency"; conv_latency "Convert latency"; conv_latency_twiddles "Convert latency (in twiddles)"; quantization "Quantization Behavior"; overflow "Overflow Behavior"; delays_bit_limit "Number bits above which to implement stage's delays in BRAM (2^? bits)"; coeffs_bit_limit "Number bits above which to store stage's coefficients in BRAM (2^? bits)"; coeff_sharing "BRAM sharing in coeff storage"; coeff_decimation "Store a fraction of coeff factors where useful"; max_fanout "Maximum fanout"; mult_spec "Multiplier impl. (0=core, 1=embedded, 2=behavioural) (left=1st stage, or just one value)"; bitgrowth "Bit growth instead of shifting"; max_bits "Max bits to growth to"; hardcode_shifts "Hardcode shift schedule"; shift_schedule "Shift schedule"; dsp48_adders "DSP48 adders in butterfly"; conv_imp_twiddles "Convert implementation in twiddles"; conv_imp "Convert implementation"
      mask help: A real-sampled biplex FFT, with output demuxed by 2.
      mask init: same as x64_15l_gonly/fft_biplex_real_2x1
      settings: AttributesFormatString=|
      | 11 stages
      | [18,18]
      | Round  (unbiased: +/- Inf)
      | Wrap
      mask Help: eval('xlWeb(''http://casper.berkeley.edu/wiki/Fft_biplex_real_2x'')')
      mask TypeOptions quantization: Truncate | Round  (unbiased: +/- Inf) | Round  (unbiased: Even Values)
      mask TypeOptions overflow: Wrap | Saturate | Error
      mask Callback hardcode_shifts:
      | hardcode_shifts = get_param(gcb, 'hardcode_shifts');
      | set_param_state(gcb, 'shift_schedule', hardcode_shifts);
      mask Callback dsp48_adders: fft_callback_dsp48_adders(gcb);
      mask TypeOptions conv_imp_twiddles: Fabric | DSP48 | Behavioural | Xilinx Cast Block
      mask TypeOptions conv_imp: Fabric | DSP48 | Behavioural | Xilinx Cast Block
  gbe_dest_ip : Subsystem  Tag=xps:sw_reg  AncestorBlock=xps_library/software register  mask(swreg){mode=one value, io_dir=From Processor, io_delay=0, sample_period=1, names=reg, bitwidths=32, arith_types=0, bin_pts=0, show_format=off}
      mask prompts: io_dir "I/O direction"; io_delay "I/O delay"; sample_period "Sample period"; names "Name:"; bitwidths "Bitwidth:"; arith_types "Type (ufix=0, fix=1, bool=2):"; bin_pts "Binary pt:"; show_format "Print format string?"
      mask init:
      | swreg_init(gcb)
      settings: AttributesFormatString=1input
      mask TypeOptions mode: one value | fields of equal size | fields of arbitrary size
      mask Callback mode: swreg_cb(gcb);
      mask TypeOptions io_dir: To Processor | From Processor
      mask Callback io_dir:
      | mask_enables = get_param(gcb, 'MaskEnables');
      | mask_names = get_param(gcb, 'MaskNames');
      | if strcmp(get_param(gcb, 'io_dir'), 'To Processor'),
      |     mask_enables{ismember(mask_names, 'sample_period')} = 'off';
      | else
      |     mask_enables{ismember(mask_names, 'sample_period')} = 'on';
      | end
      | set_param(gcb, 'MaskEnables', mask_enables);
      mask Callback bitwidths:
      | blk = gcb;
      | mode = get_param(blk, 'mode');
      | current_widths = eval(get_param(blk, 'bitwidths'));
      | if (strcmp(mode, 'one value') || strcmp(mode, 'fields of equal size')) && (length(current_widths) > 1),
      |     error('Only one width may be specified for this mode.');
      | elseif strcmp(mode, 'fields of arbitrary size')
      |     current_names = textscan(strtrim(strrep(strrep(get_param(blk, 'names'), ']', ''), '[', '')), '%s');
      |     current_names = current_names{1};
      |     numios = length(current_names);
      |     if length(current_widths) ~= numios,
      |         error('%d field names specified, but %d widths?', numios, length(current_widths));
      |     end
      | end
      | total_width = 0;
      | for ctr = 1 : length(current_widths),
      |     total_width = total_width + current_widths(ctr);
      | end
      | if total_width > 32,
      |     error('Total width must be 32 or less, set to %d.', total_width);
      | end
      mask Callback arith_types:
      | blk = gcb;
      | mode = get_param(blk, 'mode');
      | current_types = eval(get_param(blk, 'arith_types'));
      | numios = length(current_types);
      | if (strcmp(mode, 'one value') || strcmp(mode, 'fields of equal size')) && (length(current_types) > 1),
      |     error('Only one type may be specified for this mode.');
      | elseif strcmp(mode, 'fields of arbitrary size')
      |     current_names = textscan(strtrim(strrep(strrep(get_param(blk, 'names'), ']', ''), '[', '')), '%s');
      |     current_names = current_names{1};
      |     numios = length(current_names);
      |     if length(current_types) ~= numios,
      |         error('%d field names specified, but %d types?', numios, length(current_types));
      |     end
      | end
      | problem = 0;
      | for ctr = 1 : numios,
      |     t = current_types(ctr);
      |     if (t < 0) || (t > 2),
      |         problem = t;
      |         ctr = numios + 1;
      |     end
      | end
      | if problem ~= 0,
      |     error('Type cannot be %i, must be 0, 1 or 2.', problem);
      | end
      mask Callback bin_pts:
      | blk = gcb;
      | mode = get_param(blk, 'mode');
      | current_bins = eval(get_param(blk, 'bin_pts'));
      | if (strcmp(mode, 'one value') || strcmp(mode, 'fields of equal size')) && (length(current_bins) > 1),
      |     error('Only one binary pt may be specified for this mode.');
      | elseif strcmp(mode, 'fields of arbitrary size')
      |     current_names = textscan(strtrim(strrep(strrep(get_param(blk, 'names'), ']', ''), '[', '')), '%s');
      |     current_names = current_names{1};
      |     numios = length(current_names);
      |     if length(current_bins) ~= numios,
      |         error('%d field names specified, but %d binary pts?', numios, length(current_bins));
      |     end
      | end
  gbe_dest_port : Subsystem  Tag=xps:sw_reg  AncestorBlock=xps_library/software register  mask(swreg){mode=one value, io_dir=From Processor, io_delay=0, sample_period=1, names=reg, bitwidths=32, arith_types=0, bin_pts=0, show_format=off}
      mask prompts: io_dir "I/O direction"; io_delay "I/O delay"; sample_period "Sample period"; names "Name:"; bitwidths "Bitwidth:"; arith_types "Type (ufix=0, fix=1, bool=2):"; bin_pts "Binary pt:"; show_format "Print format string?"
      mask init:
      | swreg_init(gcb)
      settings: AttributesFormatString=1input
      mask TypeOptions mode: one value | fields of equal size | fields of arbitrary size
      mask Callback mode: swreg_cb(gcb);
      mask TypeOptions io_dir: To Processor | From Processor
      mask Callback io_dir:
      | mask_enables = get_param(gcb, 'MaskEnables');
      | mask_names = get_param(gcb, 'MaskNames');
      | if strcmp(get_param(gcb, 'io_dir'), 'To Processor'),
      |     mask_enables{ismember(mask_names, 'sample_period')} = 'off';
      | else
      |     mask_enables{ismember(mask_names, 'sample_period')} = 'on';
      | end
      | set_param(gcb, 'MaskEnables', mask_enables);
      mask Callback bitwidths:
      | blk = gcb;
      | mode = get_param(blk, 'mode');
      | current_widths = eval(get_param(blk, 'bitwidths'));
      | if (strcmp(mode, 'one value') || strcmp(mode, 'fields of equal size')) && (length(current_widths) > 1),
      |     error('Only one width may be specified for this mode.');
      | elseif strcmp(mode, 'fields of arbitrary size')
      |     current_names = textscan(strtrim(strrep(strrep(get_param(blk, 'names'), ']', ''), '[', '')), '%s');
      |     current_names = current_names{1};
      |     numios = length(current_names);
      |     if length(current_widths) ~= numios,
      |         error('%d field names specified, but %d widths?', numios, length(current_widths));
      |     end
      | end
      | total_width = 0;
      | for ctr = 1 : length(current_widths),
      |     total_width = total_width + current_widths(ctr);
      | end
      | if total_width > 32,
      |     error('Total width must be 32 or less, set to %d.', total_width);
      | end
      mask Callback arith_types:
      | blk = gcb;
      | mode = get_param(blk, 'mode');
      | current_types = eval(get_param(blk, 'arith_types'));
      | numios = length(current_types);
      | if (strcmp(mode, 'one value') || strcmp(mode, 'fields of equal size')) && (length(current_types) > 1),
      |     error('Only one type may be specified for this mode.');
      | elseif strcmp(mode, 'fields of arbitrary size')
      |     current_names = textscan(strtrim(strrep(strrep(get_param(blk, 'names'), ']', ''), '[', '')), '%s');
      |     current_names = current_names{1};
      |     numios = length(current_names);
      |     if length(current_types) ~= numios,
      |         error('%d field names specified, but %d types?', numios, length(current_types));
      |     end
      | end
      | problem = 0;
      | for ctr = 1 : numios,
      |     t = current_types(ctr);
      |     if (t < 0) || (t > 2),
      |         problem = t;
      |         ctr = numios + 1;
      |     end
      | end
      | if problem ~= 0,
      |     error('Type cannot be %i, must be 0, 1 or 2.', problem);
      | end
      mask Callback bin_pts:
      | blk = gcb;
      | mode = get_param(blk, 'mode');
      | current_bins = eval(get_param(blk, 'bin_pts'));
      | if (strcmp(mode, 'one value') || strcmp(mode, 'fields of equal size')) && (length(current_bins) > 1),
      |     error('Only one binary pt may be specified for this mode.');
      | elseif strcmp(mode, 'fields of arbitrary size')
      |     current_names = textscan(strtrim(strrep(strrep(get_param(blk, 'names'), ']', ''), '[', '')), '%s');
      |     current_names = current_names{1};
      |     numios = length(current_names);
      |     if length(current_bins) ~= numios,
      |         error('%d field names specified, but %d binary pts?', numios, length(current_bins));
      |     end
      | end
  gbe_en : Subsystem  Tag=xps:sw_reg  AncestorBlock=xps_library/software register  mask(swreg){mode=one value, io_dir=From Processor, io_delay=0, sample_period=1, names=reg, bitwidths=32, arith_types=0, bin_pts=0, show_format=off}
      mask prompts: io_dir "I/O direction"; io_delay "I/O delay"; sample_period "Sample period"; names "Name:"; bitwidths "Bitwidth:"; arith_types "Type (ufix=0, fix=1, bool=2):"; bin_pts "Binary pt:"; show_format "Print format string?"
      mask init:
      | swreg_init(gcb)
      settings: AttributesFormatString=1input
      mask TypeOptions mode: one value | fields of equal size | fields of arbitrary size
      mask Callback mode: swreg_cb(gcb);
      mask TypeOptions io_dir: To Processor | From Processor
      mask Callback io_dir:
      | mask_enables = get_param(gcb, 'MaskEnables');
      | mask_names = get_param(gcb, 'MaskNames');
      | if strcmp(get_param(gcb, 'io_dir'), 'To Processor'),
      |     mask_enables{ismember(mask_names, 'sample_period')} = 'off';
      | else
      |     mask_enables{ismember(mask_names, 'sample_period')} = 'on';
      | end
      | set_param(gcb, 'MaskEnables', mask_enables);
      mask Callback bitwidths:
      | blk = gcb;
      | mode = get_param(blk, 'mode');
      | current_widths = eval(get_param(blk, 'bitwidths'));
      | if (strcmp(mode, 'one value') || strcmp(mode, 'fields of equal size')) && (length(current_widths) > 1),
      |     error('Only one width may be specified for this mode.');
      | elseif strcmp(mode, 'fields of arbitrary size')
      |     current_names = textscan(strtrim(strrep(strrep(get_param(blk, 'names'), ']', ''), '[', '')), '%s');
      |     current_names = current_names{1};
      |     numios = length(current_names);
      |     if length(current_widths) ~= numios,
      |         error('%d field names specified, but %d widths?', numios, length(current_widths));
      |     end
      | end
      | total_width = 0;
      | for ctr = 1 : length(current_widths),
      |     total_width = total_width + current_widths(ctr);
      | end
      | if total_width > 32,
      |     error('Total width must be 32 or less, set to %d.', total_width);
      | end
      mask Callback arith_types:
      | blk = gcb;
      | mode = get_param(blk, 'mode');
      | current_types = eval(get_param(blk, 'arith_types'));
      | numios = length(current_types);
      | if (strcmp(mode, 'one value') || strcmp(mode, 'fields of equal size')) && (length(current_types) > 1),
      |     error('Only one type may be specified for this mode.');
      | elseif strcmp(mode, 'fields of arbitrary size')
      |     current_names = textscan(strtrim(strrep(strrep(get_param(blk, 'names'), ']', ''), '[', '')), '%s');
      |     current_names = current_names{1};
      |     numios = length(current_names);
      |     if length(current_types) ~= numios,
      |         error('%d field names specified, but %d types?', numios, length(current_types));
      |     end
      | end
      | problem = 0;
      | for ctr = 1 : numios,
      |     t = current_types(ctr);
      |     if (t < 0) || (t > 2),
      |         problem = t;
      |         ctr = numios + 1;
      |     end
      | end
      | if problem ~= 0,
      |     error('Type cannot be %i, must be 0, 1 or 2.', problem);
      | end
      mask Callback bin_pts:
      | blk = gcb;
      | mode = get_param(blk, 'mode');
      | current_bins = eval(get_param(blk, 'bin_pts'));
      | if (strcmp(mode, 'one value') || strcmp(mode, 'fields of equal size')) && (length(current_bins) > 1),
      |     error('Only one binary pt may be specified for this mode.');
      | elseif strcmp(mode, 'fields of arbitrary size')
      |     current_names = textscan(strtrim(strrep(strrep(get_param(blk, 'names'), ']', ''), '[', '')), '%s');
      |     current_names = current_names{1};
      |     numios = length(current_names);
      |     if length(current_bins) ~= numios,
      |         error('%d field names specified, but %d binary pts?', numios, length(current_bins));
      |     end
      | end
  gbe_eof : Subsystem  Tag=xps:sw_reg  AncestorBlock=xps_library/software register  mask(swreg){mode=one value, io_dir=To Processor, io_delay=0, sample_period=1, names=reg, bitwidths=32, arith_types=0, bin_pts=0, show_format=off}
      mask prompts: io_dir "I/O direction"; io_delay "I/O delay"; sample_period "Sample period"; names "Name:"; bitwidths "Bitwidth:"; arith_types "Type (ufix=0, fix=1, bool=2):"; bin_pts "Binary pt:"; show_format "Print format string?"
      mask init:
      | swreg_init(gcb)
      settings: AttributesFormatString=1output
      mask TypeOptions mode: one value | fields of equal size | fields of arbitrary size
      mask Callback mode: swreg_cb(gcb);
      mask TypeOptions io_dir: To Processor | From Processor
      mask Callback io_dir:
      | mask_enables = get_param(gcb, 'MaskEnables');
      | mask_names = get_param(gcb, 'MaskNames');
      | if strcmp(get_param(gcb, 'io_dir'), 'To Processor'),
      |     mask_enables{ismember(mask_names, 'sample_period')} = 'off';
      | else
      |     mask_enables{ismember(mask_names, 'sample_period')} = 'on';
      | end
      | set_param(gcb, 'MaskEnables', mask_enables);
      mask Callback bitwidths:
      | blk = gcb;
      | mode = get_param(blk, 'mode');
      | current_widths = eval(get_param(blk, 'bitwidths'));
      | if (strcmp(mode, 'one value') || strcmp(mode, 'fields of equal size')) && (length(current_widths) > 1),
      |     error('Only one width may be specified for this mode.');
      | elseif strcmp(mode, 'fields of arbitrary size')
      |     current_names = textscan(strtrim(strrep(strrep(get_param(blk, 'names'), ']', ''), '[', '')), '%s');
      |     current_names = current_names{1};
      |     numios = length(current_names);
      |     if length(current_widths) ~= numios,
      |         error('%d field names specified, but %d widths?', numios, length(current_widths));
      |     end
      | end
      | total_width = 0;
      | for ctr = 1 : length(current_widths),
      |     total_width = total_width + current_widths(ctr);
      | end
      | if total_width > 32,
      |     error('Total width must be 32 or less, set to %d.', total_width);
      | end
      mask Callback arith_types:
      | blk = gcb;
      | mode = get_param(blk, 'mode');
      | current_types = eval(get_param(blk, 'arith_types'));
      | numios = length(current_types);
      | if (strcmp(mode, 'one value') || strcmp(mode, 'fields of equal size')) && (length(current_types) > 1),
      |     error('Only one type may be specified for this mode.');
      | elseif strcmp(mode, 'fields of arbitrary size')
      |     current_names = textscan(strtrim(strrep(strrep(get_param(blk, 'names'), ']', ''), '[', '')), '%s');
      |     current_names = current_names{1};
      |     numios = length(current_names);
      |     if length(current_types) ~= numios,
      |         error('%d field names specified, but %d types?', numios, length(current_types));
      |     end
      | end
      | problem = 0;
      | for ctr = 1 : numios,
      |     t = current_types(ctr);
      |     if (t < 0) || (t > 2),
      |         problem = t;
      |         ctr = numios + 1;
      |     end
      | end
      | if problem ~= 0,
      |     error('Type cannot be %i, must be 0, 1 or 2.', problem);
      | end
      mask Callback bin_pts:
      | blk = gcb;
      | mode = get_param(blk, 'mode');
      | current_bins = eval(get_param(blk, 'bin_pts'));
      | if (strcmp(mode, 'one value') || strcmp(mode, 'fields of equal size')) && (length(current_bins) > 1),
      |     error('Only one binary pt may be specified for this mode.');
      | elseif strcmp(mode, 'fields of arbitrary size')
      |     current_names = textscan(strtrim(strrep(strrep(get_param(blk, 'names'), ']', ''), '[', '')), '%s');
      |     current_names = current_names{1};
      |     numios = length(current_names);
      |     if length(current_bins) ~= numios,
      |         error('%d field names specified, but %d binary pts?', numios, length(current_bins));
      |     end
      | end
  gbe_rst : Subsystem  Tag=xps:sw_reg  AncestorBlock=xps_library/software register  mask(swreg){mode=one value, io_dir=From Processor, io_delay=0, sample_period=1, names=reg, bitwidths=32, arith_types=0, bin_pts=0, show_format=off}
      mask prompts: io_dir "I/O direction"; io_delay "I/O delay"; sample_period "Sample period"; names "Name:"; bitwidths "Bitwidth:"; arith_types "Type (ufix=0, fix=1, bool=2):"; bin_pts "Binary pt:"; show_format "Print format string?"
      mask init:
      | swreg_init(gcb)
      settings: AttributesFormatString=1input
      mask TypeOptions mode: one value | fields of equal size | fields of arbitrary size
      mask Callback mode: swreg_cb(gcb);
      mask TypeOptions io_dir: To Processor | From Processor
      mask Callback io_dir:
      | mask_enables = get_param(gcb, 'MaskEnables');
      | mask_names = get_param(gcb, 'MaskNames');
      | if strcmp(get_param(gcb, 'io_dir'), 'To Processor'),
      |     mask_enables{ismember(mask_names, 'sample_period')} = 'off';
      | else
      |     mask_enables{ismember(mask_names, 'sample_period')} = 'on';
      | end
      | set_param(gcb, 'MaskEnables', mask_enables);
      mask Callback bitwidths:
      | blk = gcb;
      | mode = get_param(blk, 'mode');
      | current_widths = eval(get_param(blk, 'bitwidths'));
      | if (strcmp(mode, 'one value') || strcmp(mode, 'fields of equal size')) && (length(current_widths) > 1),
      |     error('Only one width may be specified for this mode.');
      | elseif strcmp(mode, 'fields of arbitrary size')
      |     current_names = textscan(strtrim(strrep(strrep(get_param(blk, 'names'), ']', ''), '[', '')), '%s');
      |     current_names = current_names{1};
      |     numios = length(current_names);
      |     if length(current_widths) ~= numios,
      |         error('%d field names specified, but %d widths?', numios, length(current_widths));
      |     end
      | end
      | total_width = 0;
      | for ctr = 1 : length(current_widths),
      |     total_width = total_width + current_widths(ctr);
      | end
      | if total_width > 32,
      |     error('Total width must be 32 or less, set to %d.', total_width);
      | end
      mask Callback arith_types:
      | blk = gcb;
      | mode = get_param(blk, 'mode');
      | current_types = eval(get_param(blk, 'arith_types'));
      | numios = length(current_types);
      | if (strcmp(mode, 'one value') || strcmp(mode, 'fields of equal size')) && (length(current_types) > 1),
      |     error('Only one type may be specified for this mode.');
      | elseif strcmp(mode, 'fields of arbitrary size')
      |     current_names = textscan(strtrim(strrep(strrep(get_param(blk, 'names'), ']', ''), '[', '')), '%s');
      |     current_names = current_names{1};
      |     numios = length(current_names);
      |     if length(current_types) ~= numios,
      |         error('%d field names specified, but %d types?', numios, length(current_types));
      |     end
      | end
      | problem = 0;
      | for ctr = 1 : numios,
      |     t = current_types(ctr);
      |     if (t < 0) || (t > 2),
      |         problem = t;
      |         ctr = numios + 1;
      |     end
      | end
      | if problem ~= 0,
      |     error('Type cannot be %i, must be 0, 1 or 2.', problem);
      | end
      mask Callback bin_pts:
      | blk = gcb;
      | mode = get_param(blk, 'mode');
      | current_bins = eval(get_param(blk, 'bin_pts'));
      | if (strcmp(mode, 'one value') || strcmp(mode, 'fields of equal size')) && (length(current_bins) > 1),
      |     error('Only one binary pt may be specified for this mode.');
      | elseif strcmp(mode, 'fields of arbitrary size')
      |     current_names = textscan(strtrim(strrep(strrep(get_param(blk, 'names'), ']', ''), '[', '')), '%s');
      |     current_names = current_names{1};
      |     numios = length(current_names);
      |     if length(current_bins) ~= numios,
      |         error('%d field names specified, but %d binary pts?', numios, length(current_bins));
      |     end
      | end
  gbe_tx : Subsystem  Tag=xps:sw_reg  AncestorBlock=xps_library/software register  mask(swreg){mode=one value, io_dir=To Processor, io_delay=0, sample_period=1, names=reg, bitwidths=32, arith_types=0, bin_pts=0, show_format=off}
      mask prompts: io_dir "I/O direction"; io_delay "I/O delay"; sample_period "Sample period"; names "Name:"; bitwidths "Bitwidth:"; arith_types "Type (ufix=0, fix=1, bool=2):"; bin_pts "Binary pt:"; show_format "Print format string?"
      mask init:
      | swreg_init(gcb)
      settings: AttributesFormatString=1output
      mask TypeOptions mode: one value | fields of equal size | fields of arbitrary size
      mask Callback mode: swreg_cb(gcb);
      mask TypeOptions io_dir: To Processor | From Processor
      mask Callback io_dir:
      | mask_enables = get_param(gcb, 'MaskEnables');
      | mask_names = get_param(gcb, 'MaskNames');
      | if strcmp(get_param(gcb, 'io_dir'), 'To Processor'),
      |     mask_enables{ismember(mask_names, 'sample_period')} = 'off';
      | else
      |     mask_enables{ismember(mask_names, 'sample_period')} = 'on';
      | end
      | set_param(gcb, 'MaskEnables', mask_enables);
      mask Callback bitwidths:
      | blk = gcb;
      | mode = get_param(blk, 'mode');
      | current_widths = eval(get_param(blk, 'bitwidths'));
      | if (strcmp(mode, 'one value') || strcmp(mode, 'fields of equal size')) && (length(current_widths) > 1),
      |     error('Only one width may be specified for this mode.');
      | elseif strcmp(mode, 'fields of arbitrary size')
      |     current_names = textscan(strtrim(strrep(strrep(get_param(blk, 'names'), ']', ''), '[', '')), '%s');
      |     current_names = current_names{1};
      |     numios = length(current_names);
      |     if length(current_widths) ~= numios,
      |         error('%d field names specified, but %d widths?', numios, length(current_widths));
      |     end
      | end
      | total_width = 0;
      | for ctr = 1 : length(current_widths),
      |     total_width = total_width + current_widths(ctr);
      | end
      | if total_width > 32,
      |     error('Total width must be 32 or less, set to %d.', total_width);
      | end
      mask Callback arith_types:
      | blk = gcb;
      | mode = get_param(blk, 'mode');
      | current_types = eval(get_param(blk, 'arith_types'));
      | numios = length(current_types);
      | if (strcmp(mode, 'one value') || strcmp(mode, 'fields of equal size')) && (length(current_types) > 1),
      |     error('Only one type may be specified for this mode.');
      | elseif strcmp(mode, 'fields of arbitrary size')
      |     current_names = textscan(strtrim(strrep(strrep(get_param(blk, 'names'), ']', ''), '[', '')), '%s');
      |     current_names = current_names{1};
      |     numios = length(current_names);
      |     if length(current_types) ~= numios,
      |         error('%d field names specified, but %d types?', numios, length(current_types));
      |     end
      | end
      | problem = 0;
      | for ctr = 1 : numios,
      |     t = current_types(ctr);
      |     if (t < 0) || (t > 2),
      |         problem = t;
      |         ctr = numios + 1;
      |     end
      | end
      | if problem ~= 0,
      |     error('Type cannot be %i, must be 0, 1 or 2.', problem);
      | end
      mask Callback bin_pts:
      | blk = gcb;
      | mode = get_param(blk, 'mode');
      | current_bins = eval(get_param(blk, 'bin_pts'));
      | if (strcmp(mode, 'one value') || strcmp(mode, 'fields of equal size')) && (length(current_bins) > 1),
      |     error('Only one binary pt may be specified for this mode.');
      | elseif strcmp(mode, 'fields of arbitrary size')
      |     current_names = textscan(strtrim(strrep(strrep(get_param(blk, 'names'), ']', ''), '[', '')), '%s');
      |     current_names = current_names{1};
      |     numios = length(current_names);
      |     if length(current_bins) ~= numios,
      |         error('%d field names specified, but %d binary pts?', numios, length(current_bins));
      |     end
      | end
  gbe_up : Subsystem  Tag=xps:sw_reg  AncestorBlock=xps_library/software register  mask(swreg){mode=one value, io_dir=To Processor, io_delay=0, sample_period=1, names=reg, bitwidths=32, arith_types=0, bin_pts=0, show_format=off}
      mask prompts: io_dir "I/O direction"; io_delay "I/O delay"; sample_period "Sample period"; names "Name:"; bitwidths "Bitwidth:"; arith_types "Type (ufix=0, fix=1, bool=2):"; bin_pts "Binary pt:"; show_format "Print format string?"
      mask init:
      | swreg_init(gcb)
      settings: AttributesFormatString=1output
      mask TypeOptions mode: one value | fields of equal size | fields of arbitrary size
      mask Callback mode: swreg_cb(gcb);
      mask TypeOptions io_dir: To Processor | From Processor
      mask Callback io_dir:
      | mask_enables = get_param(gcb, 'MaskEnables');
      | mask_names = get_param(gcb, 'MaskNames');
      | if strcmp(get_param(gcb, 'io_dir'), 'To Processor'),
      |     mask_enables{ismember(mask_names, 'sample_period')} = 'off';
      | else
      |     mask_enables{ismember(mask_names, 'sample_period')} = 'on';
      | end
      | set_param(gcb, 'MaskEnables', mask_enables);
      mask Callback bitwidths:
      | blk = gcb;
      | mode = get_param(blk, 'mode');
      | current_widths = eval(get_param(blk, 'bitwidths'));
      | if (strcmp(mode, 'one value') || strcmp(mode, 'fields of equal size')) && (length(current_widths) > 1),
      |     error('Only one width may be specified for this mode.');
      | elseif strcmp(mode, 'fields of arbitrary size')
      |     current_names = textscan(strtrim(strrep(strrep(get_param(blk, 'names'), ']', ''), '[', '')), '%s');
      |     current_names = current_names{1};
      |     numios = length(current_names);
      |     if length(current_widths) ~= numios,
      |         error('%d field names specified, but %d widths?', numios, length(current_widths));
      |     end
      | end
      | total_width = 0;
      | for ctr = 1 : length(current_widths),
      |     total_width = total_width + current_widths(ctr);
      | end
      | if total_width > 32,
      |     error('Total width must be 32 or less, set to %d.', total_width);
      | end
      mask Callback arith_types:
      | blk = gcb;
      | mode = get_param(blk, 'mode');
      | current_types = eval(get_param(blk, 'arith_types'));
      | numios = length(current_types);
      | if (strcmp(mode, 'one value') || strcmp(mode, 'fields of equal size')) && (length(current_types) > 1),
      |     error('Only one type may be specified for this mode.');
      | elseif strcmp(mode, 'fields of arbitrary size')
      |     current_names = textscan(strtrim(strrep(strrep(get_param(blk, 'names'), ']', ''), '[', '')), '%s');
      |     current_names = current_names{1};
      |     numios = length(current_names);
      |     if length(current_types) ~= numios,
      |         error('%d field names specified, but %d types?', numios, length(current_types));
      |     end
      | end
      | problem = 0;
      | for ctr = 1 : numios,
      |     t = current_types(ctr);
      |     if (t < 0) || (t > 2),
      |         problem = t;
      |         ctr = numios + 1;
      |     end
      | end
      | if problem ~= 0,
      |     error('Type cannot be %i, must be 0, 1 or 2.', problem);
      | end
      mask Callback bin_pts:
      | blk = gcb;
      | mode = get_param(blk, 'mode');
      | current_bins = eval(get_param(blk, 'bin_pts'));
      | if (strcmp(mode, 'one value') || strcmp(mode, 'fields of equal size')) && (length(current_bins) > 1),
      |     error('Only one binary pt may be specified for this mode.');
      | elseif strcmp(mode, 'fields of arbitrary size')
      |     current_names = textscan(strtrim(strrep(strrep(get_param(blk, 'names'), ']', ''), '[', '')), '%s');
      |     current_names = current_names{1};
      |     numios = length(current_names);
      |     if length(current_bins) ~= numios,
      |         error('%d field names specified, but %d binary pts?', numios, length(current_bins));
      |     end
      | end
  gpio_a_oen : xps_library/gpio  Tag=xps:gpio  io_group=ROACH:gpioa_oe_n  io_dir=out  arith_type=Boolean  bitwidth=1  bin_pt=0  bit_index=0  sample_period=1  use_single_ended=off  use_ddr=off  reg_iob=on  reg_clk_phase=0  termination=Pulldown
  led1 : xps_library/gpio  Tag=xps:gpio  io_group=ROACH:gpiob  io_dir=out  arith_type=Boolean  bitwidth=1  bin_pt=0  bit_index=1  sample_period=1  use_single_ended=off  use_ddr=off  reg_iob=on  reg_clk_phase=0  termination=Pulldown
  led2 : xps_library/gpio  Tag=xps:gpio  io_group=ROACH:gpiob  io_dir=out  arith_type=Boolean  bitwidth=1  bin_pt=0  bit_index=2  sample_period=1  use_single_ended=off  use_ddr=off  reg_iob=on  reg_clk_phase=0  termination=Pulldown
  led3 : xps_library/gpio  Tag=xps:gpio  io_group=ROACH:gpiob  io_dir=out  arith_type=Boolean  bitwidth=1  bin_pt=0  bit_index=3  sample_period=1  use_single_ended=off  use_ddr=off  reg_iob=on  reg_clk_phase=0  termination=Pulldown
  negedge : Subsystem  AncestorBlock=casper_library_misc/edge_detect  mask(edge_detect){edge=Falling, polarity=Active High, x_in=[0 0.08 0.08 0.16 0.16 0.24 0.24 0.32 0.32 0.4], y_in=[-1 -1  1  1  1  1  1  1  1  1], x_out=[0.6 0.68 0.68 0.76 0.76 0.84 0.84 0.92 0.92 1], y_out=[-1 -1  1  1 -1 -1 -1 -1 -1 -1]}
      mask prompts: edge "Edge Type"; polarity "Output Polarity"; x_in "Input X Positions"; y_in "Input Y Positions"; x_out "Output X Positions"; y_out "Output Y Positions"
      mask help: Output is active for one-cycle after each edge of the specified type (i.e. rising, falling or both).
      mask init: same as x64_15l_gonly/edge_detect
      settings: AttributesFormatString=|
      | falling edges
      | active high
      mask Help: Output is active for one-cycle after each edge of the specified type (i.e. rising, falling, or both).  Latency is zero.
      mask TypeOptions edge: Rising | Falling | Both
      mask TypeOptions polarity: Active High | Active Low
      mask Display:
      | plot(x_in_num,0.5+y_in_num*0.2);
      | plot(x_out_num,0.5+y_out_num*0.2);
  never{,1..3,5..6,10} (7 alike) : xbsIndex_r4/Constant  const=0  gui_display_data_type=Fixed-point  arith_type=Boolean  n_bits=16  bin_pt=14  preci_type=Single  exp_width=8  frac_width=24  explicit_period=on  period=1  equ=P=C  opselect=C  inp2=PCIN>>17  opr=+  inp1=P  carry=CIN  dbl_ovrd=off  block_type=constant
      settings: block_version=11.4
  never7 : xbsIndex_r4/Constant  const=0  gui_display_data_type=Fixed-point  arith_type=Unsigned  n_bits=16  bin_pt=0  preci_type=Single  exp_width=8  frac_width=24  explicit_period=on  period=1  equ=P=C  opselect=C  inp2=PCIN>>17  opr=+  inp1=P  carry=CIN  dbl_ovrd=off  block_type=constant
      settings: block_version=11.4
  never8 : xbsIndex_r4/Constant  const=0  gui_display_data_type=Fixed-point  arith_type=Unsigned  n_bits=32  bin_pt=0  preci_type=Single  exp_width=8  frac_width=24  explicit_period=on  period=1  equ=P=C  opselect=C  inp2=PCIN>>17  opr=+  inp1=P  carry=CIN  dbl_ovrd=off  block_type=constant
      settings: block_version=11.4
  not_zero : Subsystem
  pfb_fir_mux : Subsystem  mask(pfb_fir_mux){PFBSize=11, mux_inputs=2, TotalTaps=4, WindowType=hamming, n_inputs=0, MakeBiplex=1, BitWidthIn=12, BitWidthOut=18, CoeffBitWidth=18, CoeffDistMem=0, add_latency=1, mult_latency=2, bram_latency=3, quantization=Round  (unbiased: Even Values), fwidth=1, specify_mult=off, mult_spec=[2                                      2]}
      mask prompts: PFBSize "Size of PFB: (2^? pnts)"; mux_inputs "Signals per Input (2^?)"; TotalTaps "Total Number of Taps:"; WindowType "Windowing Function:"; n_inputs "Number of Simultaneous Inputs: (2^?)"; MakeBiplex "Make Biplex"; BitWidthIn "Input Bitwidth:"; BitWidthOut "Output Bitwidth:"; CoeffBitWidth "Coefficient Bitwidth:"; CoeffDistMem "Use Distributed Memory for Coeffs"; add_latency "Add Latency"; mult_latency "Mult Latency"; bram_latency "BRAM Latency"; quantization "Quantization Behavior"; fwidth "Bin Width Scaling (normal=1)"; specify_mult "Specify multiplier use (behavioral if not specified)"; mult_spec "Multiplier specification (0=core, 1=embedded, 2=behavioural) (left=1st tap)"
      mask init:
      | pfb_fir_mux_init(gcb, ...
      |     'PFBSize', PFBSize, ...
      |     'mux_inputs', mux_inputs, ...
      |     'TotalTaps', TotalTaps, ...
      |     'WindowType', WindowType, ...
      |     'n_inputs', n_inputs, ...
      |     'MakeBiplex', MakeBiplex, ...
      |     'BitWidthIn', BitWidthIn, ...
      |     'BitWidthOut', BitWidthOut, ...
      |     'CoeffBitWidth', CoeffBitWidth, ...
      |     'CoeffDistMem', CoeffDistMem, ...
      |     'add_latency', add_latency, ...
      |     'mult_latency', mult_latency, ...
      |     'bram_latency', bram_latency, ...
      |     'quantization', quantization, ...
      |     'fwidth', fwidth,...
      |     'specify_mult', specify_mult,...
      |     'mult_spec', mult_spec);
      settings: AttributesFormatString=taps=4, add_latency=1
      mask Help: eval('xlWeb(''http://casper.berkeley.edu/wiki/Pfb_fir'')')
      mask Callback TotalTaps:
      | %num_taps = eval(get_param(gcb, 'TotalTaps'));
      | %old_vec = eval(get_param(gcb, 'mult_spec'));
      | 
      | %vec = 2.*ones(1,num_taps);
      | %old_size = length(old_vec);
      | 
      | %if(old_size <= num_taps),
      | %   new_size = old_size;
      | %else,
      | %    new_size = num_taps;
      | %end
      | 
      | %for n = 1:new_size, vec(n) = old_vec(n); end
      | %set_param(gcb, 'mult_spec', mat2str(vec));
      mask TypeOptions WindowType: bartlett | barthannwin | blackman | blackmanharris | bohamwin | chebwin | flattopwin | gausswin | hamming | hann | kaiser | nuttallwin | parzenwin | rectwin | tukeywin | triang | userwindow
      mask TypeOptions quantization: Truncate | Round  (unbiased: +/- Inf) | Round  (unbiased: Even Values)
      mask Callback fwidth:
      | %num_taps = eval(get_param(gcb, 'TotalTaps'));
      | %old_vec = eval(get_param(gcb, 'mult_spec'));
      | 
      | %vec = 2.*ones(1,num_taps);
      | %old_size = length(old_vec);
      | 
      | %if(old_size <= num_taps),
      | %    new_size = old_size;
      | %else,
      | %    new_size = num_taps;
      | %end
      | 
      | %for n = 1:new_size, vec(n) = old_vec(n); end
      | %set_param(gcb, 'mult_spec', mat2str(vec));
      mask Callback specify_mult:
      | %specify_mult = get_param(gcb,'specify_mult');
      | %if( strcmp(specify_mult,'off')),
      | %    set_param(gcb, 'MaskEnables', {'on','on','on','on','on','on','on','on','on','on','on','on','on','on','on','off'});
      | %else
      | %    set_param(gcb, 'MaskEnables', {'on','on','on','on','on','on','on','on','on','on','on','on','on','on','on','on'});
      | %end
      mask Callback mult_spec:
      | %specify_mult = get_param(gcb,'specify_mult');
      | %if( strcmp(specify_mult,'off')),
      | %    set_param(gcb, 'MaskEnables', {'on','on','on','on','on','on','on','on','on','on','on','on','on','on','on','off'});
      | %else
      | %    set_param(gcb, 'MaskEnables', {'on','on','on','on','on','on','on','on','on','on','on','on','on','on','on','on'});
      | %end
  pfb_fir_mux1 : Subsystem  mask(pfb_fir_mux){PFBSize=11, mux_inputs=2, TotalTaps=4, WindowType=hamming, n_inputs=0, MakeBiplex=1, BitWidthIn=12, BitWidthOut=18, CoeffBitWidth=18, CoeffDistMem=0, add_latency=1, mult_latency=2, bram_latency=3, quantization=Round  (unbiased: Even Values), fwidth=1, specify_mult=off, mult_spec=[2                                      2]}
      mask prompts: PFBSize "Size of PFB: (2^? pnts)"; mux_inputs "Signals per Input (2^?)"; TotalTaps "Total Number of Taps:"; WindowType "Windowing Function:"; n_inputs "Number of Simultaneous Inputs: (2^?)"; MakeBiplex "Make Biplex"; BitWidthIn "Input Bitwidth:"; BitWidthOut "Output Bitwidth:"; CoeffBitWidth "Coefficient Bitwidth:"; CoeffDistMem "Use Distributed Memory for Coeffs"; add_latency "Add Latency"; mult_latency "Mult Latency"; bram_latency "BRAM Latency"; quantization "Quantization Behavior"; fwidth "Bin Width Scaling (normal=1)"; specify_mult "Specify multiplier use (behavioral if not specified)"; mult_spec "Multiplier specification (0=core, 1=embedded, 2=behavioural) (left=1st tap)"
      mask init: same as x64_15l_gonly/pfb_fir_mux
      settings: AttributesFormatString=taps=4, add_latency=1
      mask Help: eval('xlWeb(''http://casper.berkeley.edu/wiki/Pfb_fir'')')
      mask Callback TotalTaps:
      | %num_taps = eval(get_param(gcb, 'TotalTaps'));
      | %old_vec = eval(get_param(gcb, 'mult_spec'));
      | 
      | %vec = 2.*ones(1,num_taps);
      | %old_size = length(old_vec);
      | 
      | %if(old_size <= num_taps),
      | %   new_size = old_size;
      | %else,
      | %    new_size = num_taps;
      | %end
      | 
      | %for n = 1:new_size, vec(n) = old_vec(n); end
      | %set_param(gcb, 'mult_spec', mat2str(vec));
      mask TypeOptions WindowType: bartlett | barthannwin | blackman | blackmanharris | bohamwin | chebwin | flattopwin | gausswin | hamming | hann | kaiser | nuttallwin | parzenwin | rectwin | tukeywin | triang | userwindow
      mask TypeOptions quantization: Truncate | Round  (unbiased: +/- Inf) | Round  (unbiased: Even Values)
      mask Callback fwidth:
      | %num_taps = eval(get_param(gcb, 'TotalTaps'));
      | %old_vec = eval(get_param(gcb, 'mult_spec'));
      | 
      | %vec = 2.*ones(1,num_taps);
      | %old_size = length(old_vec);
      | 
      | %if(old_size <= num_taps),
      | %    new_size = old_size;
      | %else,
      | %    new_size = num_taps;
      | %end
      | 
      | %for n = 1:new_size, vec(n) = old_vec(n); end
      | %set_param(gcb, 'mult_spec', mat2str(vec));
      mask Callback specify_mult:
      | %specify_mult = get_param(gcb,'specify_mult');
      | %if( strcmp(specify_mult,'off')),
      | %    set_param(gcb, 'MaskEnables', {'on','on','on','on','on','on','on','on','on','on','on','on','on','on','on','off'});
      | %else
      | %    set_param(gcb, 'MaskEnables', {'on','on','on','on','on','on','on','on','on','on','on','on','on','on','on','on'});
      | %end
      mask Callback mult_spec:
      | %specify_mult = get_param(gcb,'specify_mult');
      | %if( strcmp(specify_mult,'off')),
      | %    set_param(gcb, 'MaskEnables', {'on','on','on','on','on','on','on','on','on','on','on','on','on','on','on','off'});
      | %else
      | %    set_param(gcb, 'MaskEnables', {'on','on','on','on','on','on','on','on','on','on','on','on','on','on','on','on'});
      | %end
  phase_EQ0 : Subsystem  mask{N=11-1+5-2-1, bram_lat=2, mult_lat=3, add_lat=2}
      mask prompts: N "number of coefficients (2^?)"; bram_lat "bram latency"; mult_lat "multiplier latency"; add_lat "adder latency"
      mask init:
      | set_param([gcb, '/coeff_bram'], 'addr_width', num2str(N));
  phase_EQ1 : Subsystem  mask{N=11-1+5-2-1, bram_lat=2, mult_lat=3, add_lat=2}
      mask prompts: N "number of coefficients (2^?)"; bram_lat "bram latency"; mult_lat "multiplier latency"; add_lat "adder latency"
      mask init:
      | set_param([gcb, '/coeff_bram'], 'addr_width', num2str(N));
  phase_EQ2 : Subsystem  mask{N=11-1+5-2-1, bram_lat=2, mult_lat=3, add_lat=2}
      mask prompts: N "number of coefficients (2^?)"; bram_lat "bram latency"; mult_lat "multiplier latency"; add_lat "adder latency"
      mask init:
      | set_param([gcb, '/coeff_bram'], 'addr_width', num2str(N));
  phase_EQ3 : Subsystem  mask{N=11-1+5-2-1, bram_lat=2, mult_lat=3, add_lat=2}
      mask prompts: N "number of coefficients (2^?)"; bram_lat "bram latency"; mult_lat "multiplier latency"; add_lat "adder latency"
      mask init:
      | set_param([gcb, '/coeff_bram'], 'addr_width', num2str(N));
  pipeline : Subsystem  AncestorBlock=casper_library_delays/pipeline  mask(pipeline){latency=1}
      mask help:
      | An explicitly laid-out delay line to avoid mapping to SRL16s
      | for use in pipelining to help achieve timing closure.
      mask init:
      | pipeline_init(gcb,'latency',latency);
      settings: AttributesFormatString=Latency = %<latency>
      mask Display:
      | port_label('input', 1, 'd');
      | port_label('output', 1, 'q');
      | disp(['Z^-', num2str(latency)]);
  pipeline102 : Subsystem  AncestorBlock=casper_library_delays/pipeline  mask(pipeline){latency=1}
      mask help:
      | An explicitly laid-out delay line to avoid mapping to SRL16s
      | for use in pipelining to help achieve timing closure.
      mask init:
      | pipeline_init(gcb,'latency',latency);
      settings: AttributesFormatString=Latency = %<latency>
      mask Display:
      | port_label('input', 1, 'd');
      | port_label('output', 1, 'q');
      | disp(['Z^-', num2str(latency)]);
  pipeline3 : Subsystem  AncestorBlock=casper_library_delays/pipeline  mask(pipeline){latency=1}
      mask help:
      | An explicitly laid-out delay line to avoid mapping to SRL16s
      | for use in pipelining to help achieve timing closure.
      mask init:
      | pipeline_init(gcb,'latency',latency);
      settings: AttributesFormatString=Latency = %<latency>
      mask Display:
      | port_label('input', 1, 'd');
      | port_label('output', 1, 'q');
      | disp(['Z^-', num2str(latency)]);
  qdr_transpose1 : Subsystem  AncestorBlock=casper_library_reorder/qdr_transpose  mask{idepth=(11-1), odepth=10, which_qdr=qdr1}
      mask prompts: idepth "Input blocksize (2^n)"; odepth "Output blocksize (2^n)"; which_qdr "QDR Chip"
      mask init:
      | set_param([gcb, '/qdr'], 'which_qdr', which_qdr);
      mask TypeOptions which_qdr: qdr0 | qdr1
  quant4 : Subsystem
  quant5 : Subsystem
  quant6 : Subsystem
  quant7 : Subsystem
  reorder : Subsystem  AncestorBlock=casper_library_reorder/reorder  mask(reorder){map=getfield( getfield( get_param( gcb,'UserData' ), 'parameters'),'map'), n_bits=0, n_inputs=1, bram_latency=2, map_latency=0, fanout_latency=0, double_buffer=0, bram_map=off}
      mask prompts: map "Output Order:"; n_bits "Data width in"; n_inputs "Number of inputs"; bram_latency "BRAM Latency"; map_latency "Map Latency"; fanout_latency "Fanout latency"; double_buffer "Double Buffer"; bram_map "Use BlockRAM for Map"
      mask init:
      | reorder_init(gcb, ...
      |     'map', map, ...
      |     'n_bits', n_bits, ...
      |     'n_inputs', n_inputs, ...
      |     'bram_latency', bram_latency, ...
      |     'map_latency', map_latency, ...
      |     'fanout_latency', fanout_latency, ...
      |     'double_buffer', double_buffer, ...
      |     'bram_map', bram_map);
      settings: AttributesFormatString=order=10
      mask Help: eval('xlWeb(''http://casper.berkeley.edu/wiki/Reorder'')')
  reorder_one_ant_a_time1 : Subsystem  mask{spec_chans=11-1, block_size=7}
      mask prompts: spec_chans "frequency channels? (2^?) (NFFT/2 for real FFTs)"; block_size "block size (2^?)"
      mask init:
      | partial_reorder = [0:2:2^block_size - 1]
      | 
      | reorder = []
      | for n = [0:1]
      |     reorder = [reorder, [partial_reorder]+n];
      | end
      | 
      | reorder
      | 
      | set_param([gcb, '/reorder'], 'map', tostring(reorder));
  ri_to_c{,1..3} (4 alike) : casper_library_misc/ri_to_c
  scale : Subsystem
  scale1 : Subsystem
  scale2 : Subsystem
  scale3 : Subsystem
  scale4 : Subsystem
  scale5 : Subsystem
  scale6 : Subsystem
  scale7 : Subsystem
  sim_sync : ox_lib/sim_sync  delay=9
  sim_sync1 : ox_lib/sim_sync  delay=10
  snap_ctrl : Subsystem  Tag=xps:sw_reg  AncestorBlock=xps_library/software register  mask(swreg){mode=one value, io_dir=From Processor, io_delay=0, sample_period=1, names=reg, bitwidths=32, arith_types=0, bin_pts=0, show_format=off}
      mask prompts: io_dir "I/O direction"; io_delay "I/O delay"; sample_period "Sample period"; names "Name:"; bitwidths "Bitwidth:"; arith_types "Type (ufix=0, fix=1, bool=2):"; bin_pts "Binary pt:"; show_format "Print format string?"
      mask init:
      | swreg_init(gcb)
      settings: AttributesFormatString=1input
      mask TypeOptions mode: one value | fields of equal size | fields of arbitrary size
      mask Callback mode: swreg_cb(gcb);
      mask TypeOptions io_dir: To Processor | From Processor
      mask Callback io_dir:
      | mask_enables = get_param(gcb, 'MaskEnables');
      | mask_names = get_param(gcb, 'MaskNames');
      | if strcmp(get_param(gcb, 'io_dir'), 'To Processor'),
      |     mask_enables{ismember(mask_names, 'sample_period')} = 'off';
      | else
      |     mask_enables{ismember(mask_names, 'sample_period')} = 'on';
      | end
      | set_param(gcb, 'MaskEnables', mask_enables);
      mask Callback bitwidths:
      | blk = gcb;
      | mode = get_param(blk, 'mode');
      | current_widths = eval(get_param(blk, 'bitwidths'));
      | if (strcmp(mode, 'one value') || strcmp(mode, 'fields of equal size')) && (length(current_widths) > 1),
      |     error('Only one width may be specified for this mode.');
      | elseif strcmp(mode, 'fields of arbitrary size')
      |     current_names = textscan(strtrim(strrep(strrep(get_param(blk, 'names'), ']', ''), '[', '')), '%s');
      |     current_names = current_names{1};
      |     numios = length(current_names);
      |     if length(current_widths) ~= numios,
      |         error('%d field names specified, but %d widths?', numios, length(current_widths));
      |     end
      | end
      | total_width = 0;
      | for ctr = 1 : length(current_widths),
      |     total_width = total_width + current_widths(ctr);
      | end
      | if total_width > 32,
      |     error('Total width must be 32 or less, set to %d.', total_width);
      | end
      mask Callback arith_types:
      | blk = gcb;
      | mode = get_param(blk, 'mode');
      | current_types = eval(get_param(blk, 'arith_types'));
      | numios = length(current_types);
      | if (strcmp(mode, 'one value') || strcmp(mode, 'fields of equal size')) && (length(current_types) > 1),
      |     error('Only one type may be specified for this mode.');
      | elseif strcmp(mode, 'fields of arbitrary size')
      |     current_names = textscan(strtrim(strrep(strrep(get_param(blk, 'names'), ']', ''), '[', '')), '%s');
      |     current_names = current_names{1};
      |     numios = length(current_names);
      |     if length(current_types) ~= numios,
      |         error('%d field names specified, but %d types?', numios, length(current_types));
      |     end
      | end
      | problem = 0;
      | for ctr = 1 : numios,
      |     t = current_types(ctr);
      |     if (t < 0) || (t > 2),
      |         problem = t;
      |         ctr = numios + 1;
      |     end
      | end
      | if problem ~= 0,
      |     error('Type cannot be %i, must be 0, 1 or 2.', problem);
      | end
      mask Callback bin_pts:
      | blk = gcb;
      | mode = get_param(blk, 'mode');
      | current_bins = eval(get_param(blk, 'bin_pts'));
      | if (strcmp(mode, 'one value') || strcmp(mode, 'fields of equal size')) && (length(current_bins) > 1),
      |     error('Only one binary pt may be specified for this mode.');
      | elseif strcmp(mode, 'fields of arbitrary size')
      |     current_names = textscan(strtrim(strrep(strrep(get_param(blk, 'names'), ']', ''), '[', '')), '%s');
      |     current_names = current_names{1};
      |     numios = length(current_names);
      |     if length(current_bins) ~= numios,
      |         error('%d field names specified, but %d binary pts?', numios, length(current_bins));
      |     end
      | end
  status : Subsystem  Tag=xps:sw_reg  mask{io_dir=To Processor, arith_type=Unsigned, bitwidth=32, bin_pt=0, sample_period=1, latency=0}
      mask prompts: io_dir "I/O direction"; arith_type "Data Type"; bitwidth "Data bitwidth"; bin_pt "Data binary point"; sample_period "Sample period"
      mask init:
      | gw_name = clear_name(gcb);
      | config.source = str2func('software_register_init');
      | config.toplevel = gcb;
      | xBlock( config, {io_dir, arith_type, bitwidth, bin_pt, ... 
      |     sample_period, gw_name, latency});
      mask TypeOptions io_dir: From Processor | To Processor
      mask TypeOptions arith_type: Unsigned | Signed  (2's comp)
  sync_gen : Subsystem  mask{period=10010*2^20}
  sync_gpio : xps_library/gpio  Tag=xps:gpio  io_group=ROACH:gpioa  io_dir=in  arith_type=Boolean  bitwidth=1  bin_pt=0  bit_index=7  sample_period=1  use_single_ended=off  use_ddr=off  reg_iob=on  reg_clk_phase=0  termination=Pullup
  sync_rate_change : Subsystem  mask{bits=10+3}
      mask prompts: bits "New sync rate: 2^? clocks?"
      mask help: Increases the sync pulses. For use in, for example, a snap block, where the snap can be triggered every 2^NFFT clocks, but the system sync may come much less frequently.
  sync_rate_change1 : Subsystem  mask{bits=10+3}
      mask prompts: bits "New sync rate: 2^? clocks?"
      mask help: Increases the sync pulses. For use in, for example, a snap block, where the snap can be triggered every 2^NFFT clocks, but the system sync may come much less frequently.
  sync_rate_change2 : Subsystem  mask{bits=10+3}
      mask prompts: bits "New sync rate: 2^? clocks?"
      mask help: Increases the sync pulses. For use in, for example, a snap block, where the snap can be triggered every 2^NFFT clocks, but the system sync may come much less frequently.
  sync_rate_change3 : Subsystem  mask{bits=10+3}
      mask prompts: bits "New sync rate: 2^? clocks?"
      mask help: Increases the sync pulses. For use in, for example, a snap block, where the snap can be triggered every 2^NFFT clocks, but the system sync may come much less frequently.
  sync_rate_change4 : Subsystem  mask{bits=10+3}
      mask prompts: bits "New sync rate: 2^? clocks?"
      mask help: Increases the sync pulses. For use in, for example, a snap block, where the snap can be triggered every 2^NFFT clocks, but the system sync may come much less frequently.
  ten_GbE : xps_library/ten_GbE  Tag=xps:tengbe  port=ROACH:2  mac_lite=on  open_phy=off  show_param=on  pre_emph=3  swing=800  fab_en=on  fab_mac=1122867  fab_ip=3231713812  fab_udp=10000  fab_gate=3231713793
  x64_adc : Subsystem  Tag=xps:x64_adc  AncestorBlock=xps_library/x64_adc  mask(x64_adc){adc_clk_rate=40, spi=off, ctrl_gpio=GPIO_B}
      mask prompts: adc_clk_rate "ADC clock rate (MHz)"; spi "Include SPI interface?"; ctrl_gpio "GPIO bank to use for control signals?"
      mask help: The ADC block converts analog inputs to digital outputs. Every clock cycle, the inputs are sampled and digitized to 8 bit binary point numbers in the range of [-1, 1) and are then output by the adc.
      mask init:
      | x64_adc_mask(gcb, 'spi', spi);
      mask Help: eval('xlWeb([getenv(''MLIB_ROOT''), ''\doc\html\sys_adc\sys_adc.html''])')
      mask TypeOptions ctrl_gpio: GPIO_A | GPIO_B
  x_snap : Subsystem
  xeng_oob_signal : Subsystem
  xeng_packetiser1 : Subsystem  mask{nwrd_bits=9, ant_bits=0}
      mask prompts: nwrd_bits "Payload length: (in 64bit words) (2^n)"; ant_bits "Number of antennas on this link (2^n)"
      mask help: Package 32 bit data into 64 bits and identify data as coming from antenna 0 or 1
  wires:
  adc_spi_ctrl/1(in_reg) -> Slice3/1
  Mux1/1 -> [adc0_3_in]
  Mux2/1 -> [adc4_7_in]
  Mux3/1 -> [adc8_11_in]
  Mux4/1 -> [adc12_15_in]
  Mux5/1 -> [adc16_19_in]
  Mux6/1 -> [adc20_23_in]
  Mux7/1 -> [adc24_27_in]
  Mux8/1 -> [adc28_31in]
  Delay8/1 -> Delay4/1, [adc_chan_sync0]
  [debug_sigs] -> Mux1/1, Mux2/1, Mux3/1, Mux4/1, Mux5/1, Mux6/1, Mux7/1, Mux8/1
  x64_adc/17(chan_sync) -> Delay8/1, Delay6/1
  x64_adc/1(dout0) -> Mux1/2
  x64_adc/3(dout2) -> Mux2/2
  x64_adc/5(dout4) -> Mux3/2
  x64_adc/7(dout6) -> Mux4/2
  x64_adc/9(dout8) -> Mux5/2
  x64_adc/11(dout10) -> Mux6/2
  x64_adc/13(dout12) -> Mux7/2
  x64_adc/15(dout14) -> Mux8/2
  [adc_chan_sync] -> Slice1/1
  Slice1/1 -> adc_sw/9(chan_sync)
  [adc_chan_sync] -> bus_expand/1(bus_in)
  bus_expand/1(msb_out8) -> Logical1/1
  bus_expand/2(out7) -> Logical1/2
  bus_expand/3(out6) -> Logical1/3
  bus_expand/4(out5) -> Logical1/4
  bus_expand/5(out4) -> Logical1/5
  bus_expand/6(out3) -> Logical1/6
  bus_expand/7(out2) -> Logical1/7
  bus_expand/8(lsb_out1) -> Logical1/8
  Logical1/1 -> Convert/1
  [sync_gen] -> Delay/1
  Delay/1 -> Logical2/1
  [adc_chan_sync] -> Slice9/1
  Slice9/1 -> Inverter/1
  Inverter/1 -> Logical2/2
  Logical2/1 -> Convert1/1
  ext22/1 -> Concat6/1, Logical8/1
  ext1/1 -> Concat6/2, Logical8/2
  Concat6/1 -> Convert14/1
  Convert/1 -> ext22/1
  Convert1/1 -> ext1/1
  Constant20/1 -> ctrl_sw/1(sim_1)
  ctrl_sw/1(in_reg) -> Slice/1, Slice4/1, Slice2/1, Slice12/1, Slice11/1, Slice14/1, Slice15/1, Slice22/1, Slice16/1
  Slice4/1 -> [arm_rst]
  Slice/1 -> [shift]
  Slice2/1 -> [sync_rst]
  sync_gen/1(sync) -> sim_sync1/1
  [arm_rst] -> sync_gen/2(arm)
  sync_gen/3(armed) -> [armed]
  Logical7/1 -> Convert11/1
  sync_gpio/1 -> negedge/1(in)
  [sync_rst] -> Logical7/2
  sim_sync1/1 -> adc_sync_align/1(sync)
  adc_sync_align/1(sync_out) -> [sync_gen]
  sync_gen/2(mrst) -> sim_sync/1
  adc_sync_align1/1(sync_out) -> [mrst]
  [adc_chan_sync] -> Slice7/1
  Slice12/1 -> [xaui_rcv_rst]
  Slice7/1 -> adc_sync_align/2(adc_sync), adc_sync_align1/2(adc_sync)
  Delay3/1 -> adc_sync_align1/1(sync)
  sim_sync/1 -> Delay3/1
  Slice11/1 -> [debug_sigs]
  [fft_sync_out] -> amp_EQ0/1(sync_in)
  [fft0_7_out] -> amp_EQ0/2(din)
  [fft_sync_out] -> amp_EQ1/1(sync_in)
  [fft8_15_out] -> amp_EQ1/2(din)
  amp_EQ0/1(dout) -> [amp_EQ_0_7_out]
  amp_EQ0/2(sync_out) -> [amp_EQ_sync_out]
  amp_EQ1/1(dout) -> [amp_EQ_8_15_out]
  [fft_sync_out] -> amp_EQ2/1(sync_in)
  [fft16_23_out] -> amp_EQ2/2(din)
  amp_EQ2/1(dout) -> [amp_EQ_16_23_out]
  [fft_sync_out] -> amp_EQ3/1(sync_in)
  [fft24_31_out] -> amp_EQ3/2(din)
  amp_EQ3/1(dout) -> [amp_EQ_24_31_out]
  amp_EQ0/3(of) -> [amp_of_0]
  amp_EQ1/3(of) -> [amp_of_1]
  amp_EQ2/3(of) -> [amp_of_2]
  amp_EQ3/3(of) -> [amp_of_3]
  phase_EQ0/1(dout) -> [phase_EQ_0_7_out]
  phase_EQ0/2(sync_out) -> [phase_EQ_sync_out]
  phase_EQ1/1(dout) -> [phase_EQ_8_15_out]
  phase_EQ2/1(dout) -> [phase_EQ_16_23_out]
  phase_EQ3/1(dout) -> [phase_EQ_24_31_out]
  [amp_EQ_sync_out] -> phase_EQ0/1(sync_in)
  [amp_EQ_0_7_out] -> phase_EQ0/2(din)
  [amp_EQ_sync_out] -> phase_EQ1/1(sync_in)
  [amp_EQ_8_15_out] -> phase_EQ1/2(din)
  [amp_EQ_sync_out] -> phase_EQ2/1(sync_in)
  [amp_EQ_16_23_out] -> phase_EQ2/2(din)
  [amp_EQ_sync_out] -> phase_EQ3/1(sync_in)
  [amp_EQ_24_31_out] -> phase_EQ3/2(din)
  Concat4/1 -> [quant_fftt]
  Constant1/1 -> [quant_x_eng]
  [phase_EQ_0_7_out] -> quant4/1(din)
  [phase_EQ_8_15_out] -> quant5/1(din)
  [phase_EQ_16_23_out] -> quant6/1(din)
  [phase_EQ_24_31_out] -> quant7/1(din)
  quant4/1(dout) -> Concat4/1
  quant5/1(dout) -> Concat4/2
  quant6/1(dout) -> Concat4/3
  quant7/1(dout) -> Concat4/4
  [amp_EQ_sync_out] -> Delay1/1
  [phase_EQ_sync_out] -> Delay2/1
  Delay2/1 -> [quant_fftt_sync]
  Delay1/1 -> [quant_x_eng_sync]
  quant4/2(of) -> [quant_of_f0]
  quant5/2(of) -> [quant_of_f1]
  quant6/2(of) -> [quant_of_f2]
  quant7/2(of) -> [quant_of_f3]
  Constant/1 -> reorder/2(en)
  qdr_transpose1/1(sync_out) -> reorder/1(sync)
  qdr_transpose1/2(q) -> Slice13/1
  reorder/1(sync_out) -> reorder_one_ant_a_time1/1(sync_in)
  reorder/3(dout0) -> reorder_one_ant_a_time1/2(din)
  reorder_one_ant_a_time1/1(sync_out) -> [reorder_X_sync_out]
  reorder_one_ant_a_time1/3(dout) -> [X_reorder_out]
  Slice13/1 -> reorder/3(din0)
  xeng_packetiser1/1(data_out) -> xeng_oob_signal/1(data_in)
  xeng_packetiser1/2(valid_out) -> xeng_oob_signal/2(valid_in)
  xeng_packetiser1/3(header_out) -> xeng_oob_signal/3(header)
  xeng_packetiser1/4(eof) -> xeng_oob_signal/4(eof), [eof]
  xeng_packetiser1/5(sync_out) -> xeng_oob_signal/5(sync)
  xeng_packetiser1/6(mrst_out) -> xeng_oob_signal/6(mrst)
  [X_reorder_out] -> xeng_packetiser1/1(data_in)
  [reorder_X_sync_out] -> xeng_packetiser1/2(sync_in)
  [mrst] -> xeng_packetiser1/3(mrst_in)
  xeng_oob_signal/1(data_out) -> [X_xaui64]
  xeng_oob_signal/3(valid_out) -> [tx_en_X]
  xeng_oob_signal/2(oob) -> [X_xaui_oob]
  Constant7/1 -> [s_xaui_of]
  Slice14/1 -> [white_noise]
  Mux9/1 -> [adc0_3_in1]
  [white_noise] -> Mux9/1, Mux10/1, Mux12/1, Mux11/1, Mux16/1, Mux13/1, Mux15/1, Mux14/1
  [adc0_3_in] -> Mux9/2
  Mux10/1 -> [adc4_7_in1]
  Mux12/1 -> [adc8_11_in1]
  Mux11/1 -> [adc12_15_in1]
  Mux16/1 -> [adc16_19_in1]
  Mux13/1 -> [adc20_23_in1]
  Mux15/1 -> [adc24_27_in1]
  Mux14/1 -> [adc28_31in1]
  [adc4_7_in] -> Mux10/2
  [adc8_11_in] -> Mux12/2
  [adc12_15_in] -> Mux11/2
  [adc16_19_in] -> Mux16/2
  [adc20_23_in] -> Mux13/2
  [adc24_27_in] -> Mux15/2
  [adc28_31in] -> Mux14/2
  [white_noise] -> edge_detect/1(in)
  Slice15/1 -> [white_noise_rst]
  Reinterpret1/1 -> Mux10/3
  Reinterpret7/1 -> Mux9/3
  Concat1/1 -> pipeline/1(d)
  [fft_of_0] -> Convert6/1
  [fft_of_1] -> Convert7/1
  [armed] -> pipeline3/1(d)
  never1/1 -> Concat1/6
  never/1 -> Concat1/8
  never2/1 -> Concat1/11
  Regster1/1 -> Concat1/10
  Regster2/1 -> Concat1/9
  Regster3/1 -> Concat1/7
  Logical5/1 -> Regster3/3, Regster3/1
  Logical3/1 -> Regster2/3, Regster2/1
  Logical4/1 -> Regster1/3, Regster1/1
  Regster8/1 -> Concat1/1
  never3/1 -> Concat1/2
  Regster6/1 -> Concat1/3
  Regster5/1 -> Concat1/4
  Regster4/1 -> Concat1/5
  never7/1 -> Regster8/1, not_zero/1(In1)
  never5/1 -> Regster6/3, Regster6/1
  never6/1 -> Regster5/3, Regster5/1
  pipeline3/1(q) -> Regster4/3, Regster4/1
  [status_rst] -> Regster2/2, Regster1/2
  [status_rst] -> Regster3/2
  [status_rst] -> Regster8/2, Regster6/2, Regster5/2, Regster4/2
  pipeline/1(q) -> Convert15/1
  not_zero/1(Out1) -> Regster8/3
  [amp_of_0] -> Convert8/1
  [amp_of_1] -> Convert9/1
  [amp_of_2] -> Convert12/1
  [amp_of_3] -> Convert13/1
  [quant_of_f0] -> Convert2/1
  [quant_of_f1] -> Convert3/1
  [quant_of_f2] -> Convert4/1
  [quant_of_f3] -> Convert5/1
  Constant13/1 -> snap_ctrl/1(sim_1)
  snap_ctrl/1(in_reg) -> x_snap/22(ctrl_reg)
  [fft_sync_out] -> sync_rate_change/1(In1)
  [fft0_7_out] -> x_snap/1(fft0)
  [fft8_15_out] -> x_snap/2(fft1)
  [fft16_23_out] -> x_snap/3(fft2)
  [fft24_31_out] -> x_snap/4(fft3)
  [amp_EQ_sync_out] -> sync_rate_change1/1(In1)
  [amp_EQ_0_7_out] -> x_snap/5(amp0)
  [amp_EQ_8_15_out] -> x_snap/6(amp1)
  [amp_EQ_16_23_out] -> x_snap/7(amp2)
  [amp_EQ_24_31_out] -> x_snap/8(amp3)
  [phase_EQ_0_7_out] -> x_snap/9(phase0)
  [phase_EQ_8_15_out] -> x_snap/10(phase1)
  [phase_EQ_16_23_out] -> x_snap/11(phase2)
  [phase_EQ_24_31_out] -> x_snap/12(phase3)
  [phase_EQ_sync_out] -> sync_rate_change2/1(In1)
  [quant_fftt] -> x_snap/13(quant0)
  sync_rate_change/1(Out1) -> x_snap/16(fft_sync)
  sync_rate_change1/1(Out1) -> x_snap/17(amp_sync)
  sync_rate_change2/1(Out1) -> x_snap/18(phase_sync)
  sync_rate_change3/1(Out1) -> x_snap/19(quant_sync)
  [quant_fftt_sync] -> sync_rate_change3/1(In1)
  [quant_x_eng] -> x_snap/14(quant1)
  never8/1 -> x_snap/15(x_transpose)
  [quant_x_eng_sync] -> sync_rate_change4/1(In1)
  never10/1 -> x_snap/21(x_transpose_sync)
  pipeline102/1(q) -> [status_rst]
  Slice22/1 -> pipeline102/1(d)
  Delay4/1 -> [adc_chan_sync]
  [fir_sync_out] -> a/1(sync)
  [fir0_3_out] -> a/2(in0)
  [fir4_7_out] -> a/3(in1)
  [fir8_11_out] -> a/4(in2)
  [fir12_15_out] -> a/5(in3)
  [fir16_19_out] -> a/6(in4)
  [fir20_23_out] -> a/7(in5)
  [fir24_27_out] -> a/8(in6)
  [fir28_31_out] -> a/9(in7)
  a/1(sync_out) -> [mux_sync_out]
  a/2(Out0) -> [mux0_3_out]
  a/3(Out1) -> [mux4_7_out]
  a/4(Out2) -> [mux8_11_out]
  a/5(Out3) -> [mux12_15_out]
  a/6(Out4) -> [mux16_19_out]
  a/7(Out5) -> [mux20_23_out]
  a/8(Out6) -> [mux24_27_out]
  a/9(Out7) -> [mux28_31_out]
  chan_reorder/1(sync_out) -> qdr_transpose1/1(sync)
  chan_reorder/2(dout) -> qdr_transpose1/2(d)
  x64_adc/16(dout15) -> Register/1
  Register/1 -> Mux8/3, Mux7/3, Mux6/3, Mux5/3, Mux4/3, Mux3/3, Mux2/3, Mux1/3
  Slice10/1 -> Register/2
  Slice16/1 -> [xeng_phasecal_mux]
  [quant_fftt] -> chan_reorder/2(din)
  [quant_fftt_sync] -> chan_reorder/1(sync)
  Delay6/1 -> Slice10/1
  [adc_chan_sync] -> bus_expand1/1(bus_in)
  bus_expand1/1(msb_out8) -> Logical6/1
  bus_expand1/2(out7) -> Logical6/2
  bus_expand1/3(out6) -> Logical6/3
  bus_expand1/4(out5) -> Logical6/4
  bus_expand1/5(out4) -> Logical6/5
  bus_expand1/6(out3) -> Logical6/6
  bus_expand1/7(out2) -> Logical6/7
  bus_expand1/8(lsb_out1) -> Logical6/8
  Logical6/1 -> Convert10/1
  ext2/1 -> Concat6/3, Inverter1/1
  Convert10/1 -> ext2/1
  sync_rate_change4/1(Out1) -> x_snap/20(quant_sync1)
  [mux_sync_out] -> Delay5/1
  [mux0_3_out] -> scale/1(In1)
  [mux8_11_out] -> scale1/1(In1)
  [mux4_7_out] -> scale2/1(In1)
  [mux12_15_out] -> scale3/1(In1)
  [mux_sync_out] -> Delay7/1
  [mux16_19_out] -> scale4/1(In1)
  [mux24_27_out] -> scale5/1(In1)
  [mux20_23_out] -> scale6/1(In1)
  [mux28_31_out] -> scale7/1(In1)
  [sync_gen] -> pfb_fir_mux/1(sync)
  [adc0_3_in1] -> ri_to_c/1
  [adc4_7_in1] -> ri_to_c/2
  ri_to_c/1 -> pfb_fir_mux/2(pol1_in1)
  ri_to_c1/1 -> pfb_fir_mux/3(pol2_in1)
  [adc8_11_in1] -> ri_to_c1/1
  [adc12_15_in1] -> ri_to_c1/2
  pfb_fir_mux/1(sync_out) -> [fir_sync_out]
  pfb_fir_mux/2(pol1_out1) -> c_to_ri/1
  pfb_fir_mux/3(pol2_out1) -> c_to_ri1/1
  c_to_ri/1 -> [fir0_3_out]
  c_to_ri/2 -> [fir4_7_out]
  c_to_ri1/1 -> [fir8_11_out]
  c_to_ri1/2 -> [fir12_15_out]
  [sync_gen] -> pfb_fir_mux1/1(sync)
  ri_to_c2/1 -> pfb_fir_mux1/2(pol1_in1)
  ri_to_c3/1 -> pfb_fir_mux1/3(pol2_in1)
  pfb_fir_mux1/2(pol1_out1) -> c_to_ri2/1
  pfb_fir_mux1/3(pol2_out1) -> c_to_ri3/1
  [adc16_19_in1] -> ri_to_c2/1
  [adc20_23_in1] -> ri_to_c2/2
  [adc24_27_in1] -> ri_to_c3/1
  [adc28_31in1] -> ri_to_c3/2
  c_to_ri2/1 -> [fir16_19_out]
  c_to_ri2/2 -> [fir20_23_out]
  c_to_ri3/1 -> [fir24_27_out]
  c_to_ri3/2 -> [fir28_31_out]
  Slice3/1 -> x64_adc/18(adc_rst)
  adc_sim_sync/1(Out1) -> x64_adc/17(sim_sync)
  negedge/1(out) -> Logical7/1
  Constant2/1 -> gpio_a_oen/1
  [sync_rst_led] -> ext3/1
  [adc_error_led] -> ext4/1
  Inverter1/1 -> Logical8/3
  Logical8/1 -> [adc_error_led]
  ext3/1 -> led1/1
  ext4/1 -> led2/1
  [sync_gen] -> ext5/1
  ext5/1 -> led3/1
  Convert11/1 -> sync_gen/1(rst), [sync_rst_led]
  Constant3/1 -> sync_gpio/1
  [adc0_3_in1] -> adc_sw/1(in0)
  [adc4_7_in1] -> adc_sw/2(in1)
  [adc8_11_in1] -> adc_sw/3(in2)
  [adc12_15_in1] -> adc_sw/4(in3)
  [adc16_19_in1] -> adc_sw/5(in4)
  [adc20_23_in1] -> adc_sw/6(in5)
  [adc24_27_in1] -> adc_sw/7(in6)
  [adc28_31in1] -> adc_sw/8(in7)
  edge_detect/1(out) -> White Gaussian Noise Generator/1, White Gaussian Noise Generator1/1, White Gaussian Noise Generator2/1, White Gaussian Noise Generator3/1, White Gaussian Noise Generator4/1, White Gaussian Noise Generator5/1, White Gaussian Noise Generator6/1, White Gaussian Noise Generator7/1
  Reinterpret2/1 -> Mux12/3
  Reinterpret3/1 -> Mux11/3
  Reinterpret4/1 -> Mux16/3
  Reinterpret5/1 -> Mux13/3
  Reinterpret6/1 -> Mux15/3
  Reinterpret8/1 -> Mux14/3
  White Gaussian Noise Generator/1 -> Reinterpret7/1
  White Gaussian Noise Generator1/1 -> Reinterpret1/1
  White Gaussian Noise Generator2/1 -> Reinterpret2/1
  White Gaussian Noise Generator3/1 -> Reinterpret3/1
  White Gaussian Noise Generator4/1 -> Reinterpret4/1
  White Gaussian Noise Generator5/1 -> Reinterpret5/1
  White Gaussian Noise Generator6/1 -> Reinterpret6/1
  White Gaussian Noise Generator7/1 -> Reinterpret8/1
  gbe_rst/1(in_reg) -> Slice5/1
  [X_xaui64] -> ten_GbE/2
  gbe_dest_ip/1(in_reg) -> ten_GbE/4
  gbe_dest_port/1(in_reg) -> ten_GbE/5
  Constant4/1 -> ten_GbE/7
  [eof] -> ten_GbE/6, Logical9/2
  Delay5/1 -> fft_biplex_real_2x2/1(sync)
  [shift] -> fft_biplex_real_2x2/2(shift)
  scale/1(Out1) -> fft_biplex_real_2x2/3(pol0_in)
  scale1/1(Out1) -> fft_biplex_real_2x2/4(pol1_in)
  scale2/1(Out1) -> fft_biplex_real_2x2/5(pol2_in)
  scale3/1(Out1) -> fft_biplex_real_2x2/6(pol3_in)
  fft_biplex_real_2x2/1(sync_out) -> [fft_sync_out]
  fft_biplex_real_2x2/2(pol02_out) -> [fft0_7_out]
  fft_biplex_real_2x2/4(of) -> [fft_of_0]
  fft_biplex_real_2x2/3(pol13_out) -> [fft8_15_out]
  Delay7/1 -> fft_biplex_real_2x1/1(sync)
  [shift] -> fft_biplex_real_2x1/2(shift)
  scale4/1(Out1) -> fft_biplex_real_2x1/3(pol0_in)
  scale5/1(Out1) -> fft_biplex_real_2x1/4(pol1_in)
  scale6/1(Out1) -> fft_biplex_real_2x1/5(pol2_in)
  scale7/1(Out1) -> fft_biplex_real_2x1/6(pol3_in)
  fft_biplex_real_2x1/1(sync_out) -> ?
  fft_biplex_real_2x1/2(pol02_out) -> [fft16_23_out]
  fft_biplex_real_2x1/3(pol13_out) -> [fft24_31_out]
  fft_biplex_real_2x1/4(of) -> [fft_of_1]
  Convert2/1 -> Logical5/1
  Convert3/1 -> Logical5/2
  Convert4/1 -> Logical5/3
  Convert5/1 -> Logical5/4
  Convert6/1 -> Logical3/1
  Convert7/1 -> Logical3/2
  Convert8/1 -> Logical4/1
  Convert9/1 -> Logical4/2
  Convert12/1 -> Logical4/3
  Convert13/1 -> Logical4/4
  Slice5/1 -> ten_GbE/1
  [tx_en_X] -> Logical/1
  gbe_en/1(in_reg) -> Slice8/1
  Slice8/1 -> Logical/2
  Logical/1 -> ten_GbE/3, Logical9/1
  Counter/1 -> gbe_eof/1(out_reg)
  Logical9/1 -> Counter/1
  Constant5/1 -> ten_GbE/8
  ten_GbE/1 -> Convert16/1
  ten_GbE/3 -> Counter1/1
  Counter1/1 -> gbe_tx/1(out_reg)
  Convert14/1 -> adc_sync_test/1(reg_out)
  Convert15/1 -> status/1(reg_out)
  Convert16/1 -> gbe_up/1(out_reg)
